simulink model "framework_sim"  (R2019b)
settings: Solver=FixedStepDiscrete  StartTime=T0  StopTime=Tf  FixedStep=Ts  EnableMultiTasking=on
model workspace (MAT data in the model file):
  aKalman : Simulink.Parameter (value not decoded)
  slipEnabler : Simulink.Parameter (value not decoded)
values from neighbouring files (symbols this model uses):
  enable_onlinePlots = 0    [main_framework.m]
  enable_zoom = 0    [main_framework.m]
  HLP_sampleTime = planner.replan_time    [main_framework.m]
  Kb = 10    [main_framework.m]
  Kd_vals = PID_Gain_Scheduling(:,4)    [main_framework.m]
  Ki_vals = PID_Gain_Scheduling(:,3)    [main_framework.m]
  Kp_vals = PID_Gain_Scheduling(:,2)    [main_framework.m]
  latContr_select = 4    [select_lateralController.m]
  mapObjects = scenario.scenario_data.mapObjects    [main_framework.m]
  N_vals = PID_Gain_Scheduling(:,5)    [main_framework.m]
  refRoute_fewPoints = referencePath_fewPoints.refRoute_fewPoints    [main_framework.m]    (also in refPath_poses_fewPoints.mat = [5 34.9682620653 63.3276365473 92.153562059 121.414282249 15; routePlanner.m = [x_cloth_refPath_fewPoints',y_cloth_refPath_fewPoints',theta)
  speed_vals_PID_sched = PID_Gain_Scheduling(:,1)    [main_framework.m]
  tau_D = vehicle_data.steering_system.tau_D    [dataAnalysis.m]    (also in main_framework.m)
  Ts = simulationPars.times.step_size    [main_framework.m]
  vehicle_data = getVehicleDataStruct()    [aeroModel.m]    (also in loadInitialConditions.m; longitSlipModel.m; main_framework.m; perfectAcker.m)
  X0 = loadInitialConditions    [main_framework.m]
undefined symbols (not defined in the file or in its folder): DiscIntNeverNeededParam, loadInitialPose
libraries: simulink_extras x16, drivingvehiclecontroller x2, simulink x1
(part 2 of 3)

== matlab function framework_sim/Vehicle Model ==
  settings: sampleTime=step_size
  data: X input size=24; dX output size=24; extra_params output size=26; torque_req input size=1; delta_req input
function [dX,extra_params] = Vehicle_model(X,torque_req,delta_req)

% ----------------------------------------------------------------
%% 10 DoF Vehicle Model of Formula SAE electric vehicle (Chimera Evoluzione)
%  author: Mattia Piccinini
%  email:  mattia.piccinini@unitn.it
%  date:   18/11/2019
%  The model is partly based on previous work done by Prof. F. Biral and
%  PhD students E. Pagot and L. De Pascali
% ----------------------------------------------------------------


% ----------------------------------------------------------------
%% INPUTS OF THE MODEL
% ----------------------------------------------------------------

% Model inputs are: 
%       - requested actuation torque torque_req in [Nm] (referred to electric 
%           motors if >0 and referred to the braking system if <0)
%       - requested steering angle at the steering wheel delta_req (in [rad])

% Classify the requested actuation torque on the basis of its sign, using 
% regularized positive and negative part functions to distinguish motor
% and braking torques
Tm_req = posPart(torque_req);
Tb_req = -negPart(torque_req);


% ----------------------------------------------------------------
%% OUTPUTS OF THE MODEL
% ----------------------------------------------------------------

% The outputs of the model are the derivatives of all vehicle states,
% collected in the dX vector, as well as some other useful extra parameters 
% to describe vehicle behavior, saved in the extra_params vector

% Empty output vectors are here initialized 
dX = zeros(24,1);  
extra_params = zeros(26,1);  


% ----------------------------------------------------------------
%% STATES OF THE MODEL
% ----------------------------------------------------------------

% The model has 24 states, collected in the X vector

u         = X(1);       % [m/s] vehicle longitudinal speed
v         = X(2);       % [m/s] vehicle lateral speed
z         = X(3);       % [m] vehicle heave (vertical movement of CoM)
Omega     = X(4);       % [rad/s] yaw rate
phi       = X(5);       % [rad] roll angle
mu        = X(6);       % [rad] pitch angle
delta     = X(7);       % [rad] steering angle (at the wheel)
alpha__rr = X(8);       % [rad] side slip angle rear right wheel
alpha__rl = X(9);       % [rad] side slip angle rear left wheel
alpha__fr = X(10);      % [rad] side slip angle front right wheel
alpha__fl = X(11);      % [rad] side slip angle front left wheel
kappa__rr = X(12);      % [-] longitudinal slip rear right wheel
kappa__rl = X(13);      % [-] longitudinal slip rear left wheel
kappa__fr = X(14);      % [-] longitudinal slip front right wheel
kappa__fl = X(15);      % [-] longitudinal slip front left wheel
omega__rr = X(16);      % [rad/s] rotational speed rear right wheel
omega__rl = X(17);      % [rad/s] rotational speed rear left wheel 
omega__fr = X(18);      % [rad/s] rotational speed front right wheel 
omega__fl = X(19);      % [rad/s] rotational speed front left wheel 
z__dot    = X(20);      % [m/s] heave rate of change
phi__dot  = X(21);      % [rad/s] roll angle rate of change
mu__dot   = X(22);      % [rad/s] pitch angle rate of change
Tm        = X(23);      % [Nm] motor torque (same for both rear motors)
Tb        = X(24);      % [Nm] brake torque (same for each wheel)


% ----------------------------------------------------------------
%% VEHICLE DATA AND PARAMETERS
% ----------------------------------------------------------------

% Load a struct containing vehicle parameters. 
% For the meaning of each parameter, refer to the file getVehicleDataStruct
params = getVehicleDataStruct; 

% ----------------------
% SUSPENSION DATA
% ----------------------
% REAR
h__rc_r =  params.rear_suspension.h_rc_r;
% FRONT
h__rc_f =  params.front_suspension.h_rc_f;

% ----------------------                                              
% CHASSIS DATA
% ----------------------
is__xx = params.chassis.is_xx;
is__yy = params.chassis.is_yy;
is__zz = params.chassis.is_zz;
is__xz = params.chassis.is_xz;

% ----------------------
% UNSPRUNG MASS DATA
% ----------------------
% REAR
Rr = params.rear_wheel.Rr;                   
iwa__r = params.rear_wheel.iwa_r;
iwa__f = iwa__r;
% FRONT
Rf = params.front_wheel.Rf;                         

% ----------------------
% OVERALL VEHICLE DATA
% ----------------------
Lf = params.vehicle.Lf;        
Lr = params.vehicle.Lr;             
h__Gs = params.vehicle.hGs;      
Wf = params.vehicle.Wf;    
Wr = params.vehicle.Wr;    
lx = params.vehicle.lx;
ly = params.vehicle.ly;
z__static = h__rc_f + Lf * ((h__rc_r - h__rc_f)/(Lf+Lr));
% Inertia and mass
m = params.vehicle.m;  
ms = params.vehicle.ms;
g = params.vehicle.g;     
i__zz = params.vehicle.i_zz;
i__xz = params.vehicle.i_xz;

% ----------------------
% STEERING SYSTEM DATA        
% ----------------------
tau__D = params.steering_system.tau_D;             
tau__H = params.steering_system.tau_H;   

% ----------------------
% TRANSMISSION DATA
% ----------------------
tau_red = params.transmission.tau_red; 
eff_red = params.transmission.eff_red;

% ----------------------
% MOTOR AND BRAKE ACTUATION DATA
% ----------------------
tau_mot = params.motor.tau_mot;
tau_br  = params.braking.tau_br;


% ----------------------------------------------------------------
%% AUXILIARY MODELS
% ----------------------------------------------------------------

% ----------------------
% MOTOR MODEL
% ----------------------
% Driving torques at the wheels
Tw__rr_traction = MotorModel(Tm,omega__rr,tau_red,eff_red);
Tw__rl_traction = MotorModel(Tm,omega__rl,tau_red,eff_red);
 
% ----------------------
% BRAKE MODEL
% ----------------------
% Rear wheels braking model
[Tw__rr_brake,Tw__rl_brake] = brakeModelRear(Tb,Tb,omega__rr,omega__rl); 
% Front wheels braking model
[Tw__fr_brake,Tw__fl_brake] = brakeModelFront(Tb,Tb,omega__fr,omega__fl);

% ----------------------
% WHEEL TORQUES
% ----------------------
% The total torque for each wheel is the algebraic sum of motor and brake torques
Tw__rr = Tw__rr_traction + Tw__rr_brake;
Tw__rl = Tw__rl_traction + Tw__rl_brake;
Tw__fr = Tw__fr_brake;
Tw__fl = Tw__fl_brake;

% ----------------------
% CAMBER MODEL
% ----------------------
% Static camber + camber gain model, as a function of roll angle phi
[gamma__rr, gamma__rl, gamma__fr, gamma__fl] = camberModel(phi);

% ----------------------
% ACKERMANN STEERING MODEL
% ----------------------
% Compute steering angles for front wheels, with perfect Ackerman steering model
[delta__fr, delta__fl] = perfectAcker(delta);

% ----------------------
% VERTICAL TIRE FORCES MODEL
% ----------------------
% Compute vertical tire loads
VerticalForces = LoadTransferModel(z,phi,mu,z__dot,phi__dot,mu__dot,Omega,u);
Fz__rr = VerticalForces.Fz_rr;
Fz__rl = VerticalForces.Fz_rl;
Fz__fr = VerticalForces.Fz_fr;
Fz__fl = VerticalForces.Fz_fl;

% ----------------------
% LONGITUDINAL SLIPS
% ----------------------
% Longitudinal slip model including a correction for low speed 
[kappa__rr_corr,kappa__rl_corr,kappa__fr_corr,kappa__fl_corr] = longitSlipModel(u,Omega,kappa__rr,kappa__rl,kappa__fr,kappa__fl,omega__rr,omega__rl,omega__fr,omega__fl,delta__fr,delta__fl,Fz__rr,Fz__rl,Fz__fr,Fz__fl,gamma__rr,gamma__rl,gamma__fr,gamma__fl,loadPacejkaParam);

% ----------------------
% AERODYNAMIC MODEL
% ----------------------
% Aero drag, downforce at rear axle, downforce at front axle
[FAxc, FAz__r, FAz__f] = aeroModel(u);
          
% ----------------------
% TIRE PACEJKA MODEL
% ----------------------
% Ensure symmetric behavior of left and right tires by calculating the
% forces and moments for left tires via a previous change of sign of the
% side slip alpha and the camber gamma
[Fx__rr,Fy__rr,AM__rr] = pacejka_model(kappa__rr_corr,Fz__rr,alpha__rr,gamma__rr,loadPacejkaParam);
[Fx__rl,Fy__rl,AM__rl] = pacejka_model(kappa__rl_corr,Fz__rl,-alpha__rl,-gamma__rl,loadPacejkaParam);
[Fx__fr,Fy__fr,AM__fr] = pacejka_model(kappa__fr_corr,Fz__fr,alpha__fr,gamma__fr,loadPacejkaParam);
[Fx__fl,Fy__fl,AM__fl] = pacejka_model(kappa__fl_corr,Fz__fl,-alpha__fl,-gamma__fl,loadPacejkaParam);
% Now perform a second change of sign in order to restore the correct operating conditions
Fy__rl = -Fy__rl; AM__rl = -AM__rl;
Fy__fl = -Fy__fl; AM__fl = -AM__fl;

% ----------------------
% STEADY STATE LONGITUDINAL SLIPS
% ----------------------
[kappa__rr_ss,kappa__rl_ss,kappa__fr_ss,kappa__fl_ss] = steadyStateLongSlips(omega__rr,omega__rl,omega__fr,omega__fl,Omega,u,delta__fr,delta__fl);


% ----------------------------------------------------------------
%% VEHICLE MODEL DIFFERENTIAL EQUATIONS
% ----------------------------------------------------------------

% The following system of ODE is imported from Maple symbolic model

% 3 Newton equations
u_Dot        = ((2 * is__xz * ((is__xx - is__yy - is__zz) * Omega ^ 2 + (h__Gs - z__static) * (-m * g + g * ms - FAz__f - FAz__r + Fz__fl + Fz__fr + Fz__rl + Fz__rr)) * (h__Gs - z__static) * (ms * (h__Gs - z__static) * (ms - m) * z - z__static * (h__Gs - z__static) * ms ^ 2 + m * z__static * (h__Gs - z__static) * ms - m * (is__xx + is__zz)) * ms * mu ^ 2) + ((2 * is__xz * (h__Gs - z__static) ^ 2 * (v * (ms - m) * Omega + delta__fl * Fy__fl + delta__fr * Fy__fr - Fx__fl - Fx__fr - Fx__rl - Fx__rr) * (ms - m) * ms ^ 2 * z ^ 2) + 0.2e1 * (((h__Gs - z__static) * (i__xz * is__xz + i__zz * (is__xx - is__yy - is__zz)) * (ms - m) * ms * Omega ^ 2) - ((ms ^ 2 * is__zz * u * (h__Gs - z__static) ^ 2 * phi) + 0.2e1 * is__xz * (-(ms * iwa__f * omega__fl * (h__Gs - z__static) * delta__fl) / 0.2e1 - (ms * iwa__f * omega__fr * (h__Gs - z__static) * delta__fr) / 0.2e1 + ((z__static * (h__Gs - z__static) * ms ^ 2) - (m * z__static * (h__Gs - z__static) * ms) + (m * (is__xx + is__yy + is__zz)) / 0.2e1) * v + (ms * phi__dot * (is__xx - is__yy - is__zz) * (h__Gs - z__static)) / 0.2e1)) * (ms - m) * Omega + (is__xz * Fy__fl * ((h__Gs - z__static) * (h__Gs - 2 * z__static) * ms ^ 2 + (-h__Gs ^ 2 * m + 3 * h__Gs * m * z__static - 2 * m * z__static ^ 2 + is__yy) * ms - m * (is__xx + is__yy + is__zz)) * delta__fl) + (is__xz * Fy__fr * ((h__Gs - z__static) * (h__Gs - 2 * z__static) * ms ^ 2 + (-h__Gs ^ 2 * m + 3 * h__Gs * m * z__static - 2 * m * z__static ^ 2 + is__yy) * ms - m * (is__xx + is__yy + is__zz)) * delta__fr) - is__xz * (((h__Gs - z__static) * (h__Gs - 2 * z__static - Rf) * ms ^ 2) + (-(2 * m * z__static ^ 2) + 0.3e1 * (h__Gs - Rf / 0.3e1) * m * z__static - (h__Gs * (h__Gs - Rf) * m) + is__yy) * ms - (m * (is__xx + is__yy + is__zz))) * Fx__fl - is__xz * (((h__Gs - z__static) * (h__Gs - 2 * z__static - Rf) * ms ^ 2) + (-(2 * m * z__static ^ 2) + 0.3e1 * (h__Gs - Rf / 0.3e1) * m * z__static - (h__Gs * (h__Gs - Rf) * m) + is__yy) * ms - (m * (is__xx + is__yy + is__zz))) * Fx__fr - is__xz * (((h__Gs - z__static) * (h__Gs - 2 * z__static - Rr) * ms ^ 2) + (-(2 * m * z__static ^ 2) + 0.3e1 * (h__Gs - Rr / 0.3e1) * m * z__static - (h__Gs * (h__Gs - Rr) * m) + is__yy) * ms - (m * (is__xx + is__yy + is__zz))) * Fx__rl - is__xz * (((h__Gs - z__static) * (h__Gs - 2 * z__static - Rr) * ms ^ 2) + (-(2 * m * z__static ^ 2) + 0.3e1 * (h__Gs - Rr / 0.3e1) * m * z__static - (h__Gs * (h__Gs - Rr) * m) + is__yy) * ms - (m * (is__xx + is__yy + is__zz))) * Fx__rr + ((ms - m) * (ms * (h__Gs - z__static) * (-Lf * is__xz + h__Gs * i__zz - i__zz * z__static) * Fz__fl + ms * (h__Gs - z__static) * (-Lf * is__xz + h__Gs * i__zz - i__zz * z__static) * Fz__fr + ms * (h__Gs - z__static) * (Lr * is__xz + h__Gs * i__zz - i__zz * z__static) * Fz__rl + ms * (h__Gs - z__static) * (Lr * is__xz + h__Gs * i__zz - i__zz * z__static) * Fz__rr - ms * (h__Gs - z__static) * (-Lf * is__xz + h__Gs * i__zz - i__zz * z__static) * FAz__f - ms * (h__Gs - z__static) * (Lr * is__xz + h__Gs * i__zz - i__zz * z__static) * FAz__r + ((h__Gs - z__static) ^ 2 * ms + is__yy) * is__xz * FAxc + (-is__xz * Tw__fl - is__xz * Tw__fr - is__xz * Tw__rl - is__xz * Tw__rr + g * i__zz * (h__Gs - z__static) * (ms - m)) * (h__Gs - z__static) * ms))) * (h__Gs - z__static) * ms * z - (2 * (h__Gs - z__static) * ((h__Gs - z__static) * z__static * (i__xz * is__xz + i__zz * (is__xx - is__yy - is__zz)) * ms ^ 2 - (h__Gs - z__static) * z__static * (i__xz * is__xz + i__zz * (is__xx - is__yy - is__zz)) * m * ms + (i__xz * (is__yy + 2 * is__zz) * is__xz + i__zz * is__xx * (is__xx - is__yy - is__zz)) * m) * ms * Omega ^ 2) + ((2 * (h__Gs - z__static) ^ 2 * is__zz * u * (z__static * (h__Gs - z__static) * ms ^ 2 - m * z__static * (h__Gs - z__static) * ms + is__xx * m) * ms ^ 2 * phi + 2 * is__xz * (-ms * iwa__f * omega__fl * (h__Gs - z__static) * delta__fl - ms * iwa__f * omega__fr * (h__Gs - z__static) * delta__fr + (z__static * (h__Gs - z__static) * ms ^ 2 - m * z__static * (h__Gs - z__static) * ms + is__yy * m) * v + ms * phi__dot * (is__xx - is__yy - is__zz) * (h__Gs - z__static)) * (z__static * (h__Gs - z__static) * ms ^ 2 - m * z__static * (h__Gs - z__static) * ms + m * (is__xx + is__zz))) * Omega) - (2 * ((h__Gs - z__static) ^ 2 * ms + is__yy) * is__xz * Fy__fl * (z__static * (h__Gs - z__static) * ms ^ 2 - m * z__static * (h__Gs - z__static) * ms + m * (is__xx + is__zz)) * delta__fl) - (2 * ((h__Gs - z__static) ^ 2 * ms + is__yy) * is__xz * Fy__fr * (z__static * (h__Gs - z__static) * ms ^ 2 - m * z__static * (h__Gs - z__static) * ms + m * (is__xx + is__zz)) * delta__fr) + (2 * ((h__Gs - z__static) * (h__Gs - z__static - Rf) * ms + is__yy) * is__xz * (z__static * (h__Gs - z__static) * ms ^ 2 - m * z__static * (h__Gs - z__static) * ms + m * (is__xx + is__zz)) * Fx__fl) + (2 * ((h__Gs - z__static) * (h__Gs - z__static - Rf) * ms + is__yy) * is__xz * (z__static * (h__Gs - z__static) * ms ^ 2 - m * z__static * (h__Gs - z__static) * ms + m * (is__xx + is__zz)) * Fx__fr) + (2 * is__xz * ((h__Gs - z__static) * (h__Gs - z__static - Rr) * ms + is__yy) * (z__static * (h__Gs - z__static) * ms ^ 2 - m * z__static * (h__Gs - z__static) * ms + m * (is__xx + is__zz)) * Fx__rl) + (2 * is__xz * ((h__Gs - z__static) * (h__Gs - z__static - Rr) * ms + is__yy) * (z__static * (h__Gs - z__static) * ms ^ 2 - m * z__static * (h__Gs - z__static) * ms + m * (is__xx + is__zz)) * Fx__rr) - (2 * (h__Gs - z__static) * (z__static * (h__Gs - z__static) * (-Lf * is__xz + h__Gs * i__zz - i__zz * z__static) * ms ^ 2 - m * z__static * (h__Gs - z__static) * (-Lf * is__xz + h__Gs * i__zz - i__zz * z__static) * ms - m * ((-i__xz * is__xz + i__zz * is__xx) * z__static + (i__xz * is__xz - i__zz * is__xx) * h__Gs + is__xz * Lf * (is__xx + is__zz))) * ms * Fz__fl) - (2 * (h__Gs - z__static) * (z__static * (h__Gs - z__static) * (-Lf * is__xz + h__Gs * i__zz - i__zz * z__static) * ms ^ 2 - m * z__static * (h__Gs - z__static) * (-Lf * is__xz + h__Gs * i__zz - i__zz * z__static) * ms - m * ((-i__xz * is__xz + i__zz * is__xx) * z__static + (i__xz * is__xz - i__zz * is__xx) * h__Gs + is__xz * Lf * (is__xx + is__zz))) * ms * Fz__fr) - (2 * (z__static * (h__Gs - z__static) * (Lr * is__xz + h__Gs * i__zz - i__zz * z__static) * ms ^ 2 - m * z__static * (h__Gs - z__static) * (Lr * is__xz + h__Gs * i__zz - i__zz * z__static) * ms - ((-i__xz * is__xz + i__zz * is__xx) * z__static + (i__xz * is__xz - i__zz * is__xx) * h__Gs - is__xz * Lr * (is__xx + is__zz)) * m) * (h__Gs - z__static) * ms * Fz__rl) - (2 * (z__static * (h__Gs - z__static) * (Lr * is__xz + h__Gs * i__zz - i__zz * z__static) * ms ^ 2 - m * z__static * (h__Gs - z__static) * (Lr * is__xz + h__Gs * i__zz - i__zz * z__static) * ms - ((-i__xz * is__xz + i__zz * is__xx) * z__static + (i__xz * is__xz - i__zz * is__xx) * h__Gs - is__xz * Lr * (is__xx + is__zz)) * m) * (h__Gs - z__static) * ms * Fz__rr) + (2 * (h__Gs - z__static) * (z__static * (h__Gs - z__static) * (-Lf * is__xz + h__Gs * i__zz - i__zz * z__static) * ms ^ 2 - m * z__static * (h__Gs - z__static) * (-Lf * is__xz + h__Gs * i__zz - i__zz * z__static) * ms - m * ((-i__xz * is__xz + i__zz * is__xx) * z__static + (i__xz * is__xz - i__zz * is__xx) * h__Gs + is__xz * Lf * (is__xx + is__zz))) * ms * FAz__f) + (2 * (z__static * (h__Gs - z__static) * (Lr * is__xz + h__Gs * i__zz - i__zz * z__static) * ms ^ 2 - m * z__static * (h__Gs - z__static) * (Lr * is__xz + h__Gs * i__zz - i__zz * z__static) * ms - ((-i__xz * is__xz + i__zz * is__xx) * z__static + (i__xz * is__xz - i__zz * is__xx) * h__Gs - is__xz * Lr * (is__xx + is__zz)) * m) * (h__Gs - z__static) * ms * FAz__r) - (2 * ((h__Gs - z__static) ^ 2 * ms + is__yy) * is__xz * (z__static * (h__Gs - z__static) * ms ^ 2 - m * z__static * (h__Gs - z__static) * ms + m * (is__xx + is__zz)) * FAxc) - (2 * (-is__xz * (z__static * (h__Gs - z__static) * ms ^ 2 - m * z__static * (h__Gs - z__static) * ms + m * (is__xx + is__zz)) * Tw__fl - is__xz * (z__static * (h__Gs - z__static) * ms ^ 2 - m * z__static * (h__Gs - z__static) * ms + m * (is__xx + is__zz)) * Tw__fr - is__xz * (z__static * (h__Gs - z__static) * ms ^ 2 - m * z__static * (h__Gs - z__static) * ms + m * (is__xx + is__zz)) * Tw__rl - is__xz * (z__static * (h__Gs - z__static) * ms ^ 2 - m * z__static * (h__Gs - z__static) * ms + m * (is__xx + is__zz)) * Tw__rr + (h__Gs - z__static) * (ms - m) * g * (i__zz * z__static * (h__Gs - z__static) * ms ^ 2 - i__zz * m * z__static * (h__Gs - z__static) * ms - m * (i__xz * is__xz - i__zz * is__xx))) * (h__Gs - z__static) * ms)) * mu + (2 * (h__Gs - z__static) ^ 2 * (v * (ms - m) * Omega + delta__fl * Fy__fl + delta__fr * Fy__fr - Fx__fl - Fx__fr - Fx__rl - Fx__rr) * (ms - m) * i__zz * ms ^ 2 * z ^ 2) - 0.4e1 * (h__Gs - z__static) * (-(ms * (is__xz * is__zz * phi ^ 2 + i__xz * i__zz) * (h__Gs - z__static) * (ms - m) * Omega ^ 2) / 0.2e1 + (-(ms * i__zz * iwa__f * omega__fl * (h__Gs - z__static) * delta__fl) / 0.2e1 - (ms * i__zz * iwa__f * omega__fr * (h__Gs - z__static) * delta__fr) / 0.2e1 + ((i__zz * z__static * (h__Gs - z__static) * ms ^ 2) - (i__zz * m * z__static * (h__Gs - z__static) * ms) - ((i__xz * is__xz - i__zz * (is__xx + is__yy)) * m) / 0.2e1) * v + (ms * i__zz * phi__dot * (is__xx - is__yy - is__zz) * (h__Gs - z__static)) / 0.2e1) * (ms - m) * Omega - ((((Lf * (h__Gs - z__static) * ms - h__Gs * m * Lf + m * z__static * Lf - is__xz) * Fx__fl) + (Fy__fl * Wf * (h__Gs - z__static) * (ms - m)) / 0.2e1) * delta__fl + (((Lf * (h__Gs - z__static) * ms - h__Gs * m * Lf + m * z__static * Lf - is__xz) * Fx__fr) - (Fy__fr * Wf * (h__Gs - z__static) * (ms - m)) / 0.2e1) * delta__fr - (Wf * (h__Gs - z__static) * (ms - m) * Fx__fl) / 0.2e1 + (Wf * (h__Gs - z__static) * (ms - m) * Fx__fr) / 0.2e1 - (Wr * (h__Gs - z__static) * (ms - m) * Fx__rl) / 0.2e1 + (Wr * (h__Gs - z__static) * (ms - m) * Fx__rr) / 0.2e1 + ((Lf * (h__Gs - z__static) * ms - h__Gs * m * Lf + m * z__static * Lf - is__xz) * Fy__fl) + ((Lf * (h__Gs - z__static) * ms - h__Gs * m * Lf + m * z__static * Lf - is__xz) * Fy__fr) + ((-Lr * (h__Gs - z__static) * ms + h__Gs * m * Lr - m * z__static * Lr - is__xz) * Fy__rl) + ((-Lr * (h__Gs - z__static) * ms + h__Gs * m * Lr - m * z__static * Lr - is__xz) * Fy__rr) + ((AM__fl + AM__fr + AM__rl + AM__rr) * (h__Gs - z__static) * (ms - m))) * is__zz * ms * phi / 0.2e1 - (Fy__fl * (i__zz * (h__Gs - z__static) * (h__Gs - 2 * z__static) * ms ^ 2 - i__zz * (h__Gs ^ 2 * m - 3 * h__Gs * m * z__static + 2 * m * z__static ^ 2 - is__yy) * ms + (i__xz * is__xz - i__zz * (is__xx + is__yy)) * m) * delta__fl) / 0.2e1 - (Fy__fr * (i__zz * (h__Gs - z__static) * (h__Gs - 2 * z__static) * ms ^ 2 - i__zz * (h__Gs ^ 2 * m - 3 * h__Gs * m * z__static + 2 * m * z__static ^ 2 - is__yy) * ms + (i__xz * is__xz - i__zz * (is__xx + is__yy)) * m) * delta__fr) / 0.2e1 + ((i__zz * (h__Gs - z__static) * (h__Gs - 2 * z__static - Rf) * ms ^ 2) / 0.2e1 - ((2 * m * z__static ^ 2) - 0.3e1 * (h__Gs - Rf / 0.3e1) * m * z__static + (h__Gs * (h__Gs - Rf) * m) - is__yy) * i__zz * ms / 0.2e1 + ((i__xz * is__xz - i__zz * (is__xx + is__yy)) * m) / 0.2e1) * Fx__fl + ((i__zz * (h__Gs - z__static) * (h__Gs - 2 * z__static - Rf) * ms ^ 2) / 0.2e1 - ((2 * m * z__static ^ 2) - 0.3e1 * (h__Gs - Rf / 0.3e1) * m * z__static + (h__Gs * (h__Gs - Rf) * m) - is__yy) * i__zz * ms / 0.2e1 + ((i__xz * is__xz - i__zz * (is__xx + is__yy)) * m) / 0.2e1) * Fx__fr + ((i__zz * (h__Gs - z__static) * (h__Gs - 2 * z__static - Rr) * ms ^ 2) / 0.2e1 - ((2 * m * z__static ^ 2) - 0.3e1 * (h__Gs - Rr / 0.3e1) * m * z__static + (h__Gs * (h__Gs - Rr) * m) - is__yy) * i__zz * ms / 0.2e1 + ((i__xz * is__xz - i__zz * (is__xx + is__yy)) * m) / 0.2e1) * Fx__rl + ((i__zz * (h__Gs - z__static) * (h__Gs - 2 * z__static - Rr) * ms ^ 2) / 0.2e1 - ((2 * m * z__static ^ 2) - 0.3e1 * (h__Gs - Rr / 0.3e1) * m * z__static + (h__Gs * (h__Gs - Rr) * m) - is__yy) * i__zz * ms / 0.2e1 + ((i__xz * is__xz - i__zz * (is__xx + is__yy)) * m) / 0.2e1) * Fx__rr - ((ms - m) * i__zz * (-Lf * (h__Gs - z__static) * ms * Fz__fl - Lf * (h__Gs - z__static) * ms * Fz__fr + Lr * (h__Gs - z__static) * ms * Fz__rl + Lr * (h__Gs - z__static) * ms * Fz__rr + Lf * (h__Gs - z__static) * ms * FAz__f - Lr * (h__Gs - z__static) * ms * FAz__r + ((h__Gs - z__static) ^ 2 * ms + is__yy) * FAxc - ms * (Tw__fl + Tw__fr + Tw__rl + Tw__rr) * (h__Gs - z__static))) / 0.2e1) * ms * z - (2 * (h__Gs - z__static) * ((z__static * (h__Gs - z__static) * ms ^ 2 - m * z__static * (h__Gs - z__static) * ms + m * (is__yy - is__zz)) * is__xz * is__zz * phi ^ 2 + i__xz * (i__zz * z__static * (h__Gs - z__static) * ms ^ 2 - i__zz * m * z__static * (h__Gs - z__static) * ms - m * (i__xz * is__xz - i__zz * is__xx))) * ms * Omega ^ 2) + ((2 * is__xz * (h__Gs - z__static) * (-iwa__f * omega__fl - iwa__f * omega__fr + (is__xx - is__yy + is__zz) * mu__dot - iwa__r * (omega__rl + omega__rr)) * is__zz * m * ms * phi + 2 * (-ms * iwa__f * omega__fl * (h__Gs - z__static) * delta__fl - ms * iwa__f * omega__fr * (h__Gs - z__static) * delta__fr + (z__static * (h__Gs - z__static) * ms ^ 2 - m * z__static * (h__Gs - z__static) * ms + is__yy * m) * v + ms * phi__dot * (is__xx - is__yy - is__zz) * (h__Gs - z__static)) * (i__zz * z__static * (h__Gs - z__static) * ms ^ 2 - i__zz * m * z__static * (h__Gs - z__static) * ms - m * (i__xz * is__xz - i__zz * is__xx))) * Omega) - (2 * ms * is__xz * is__zz * m * (h__Gs - z__static) ^ 2 * (-m * g + g * ms - FAz__f - FAz__r + Fz__fl + Fz__fr + Fz__rl + Fz__rr) * phi ^ 2) - 0.2e1 * (h__Gs - z__static) * ((((z__static * Lf * (h__Gs - z__static) * ms ^ 2 - z__static * (h__Gs * m * Lf - m * z__static * Lf + is__xz) * ms + m * (is__xx * Lf - is__xz * Rf + h__Gs * is__xz)) * Fx__fl) + (Wf * (z__static * (h__Gs - z__static) * ms ^ 2 - m * z__static * (h__Gs - z__static) * ms + is__xx * m) * Fy__fl) / 0.2e1 + (is__xz * m * Tw__fl)) * delta__fl + (((z__static * Lf * (h__Gs - z__static) * ms ^ 2 - z__static * (h__Gs * m * Lf - m * z__static * Lf + is__xz) * ms + m * (is__xx * Lf - is__xz * Rf + h__Gs * is__xz)) * Fx__fr) - (Wf * (z__static * (h__Gs - z__static) * ms ^ 2 - m * z__static * (h__Gs - z__static) * ms + is__xx * m) * Fy__fr) / 0.2e1 + (is__xz * m * Tw__fr)) * delta__fr - (Wf * (z__static * (h__Gs - z__static) * ms ^ 2 - m * z__static * (h__Gs - z__static) * ms + is__xx * m) * Fx__fl) / 0.2e1 + (Wf * (z__static * (h__Gs - z__static) * ms ^ 2 - m * z__static * (h__Gs - z__static) * ms + is__xx * m) * Fx__fr) / 0.2e1 - (Wr * (z__static * (h__Gs - z__static) * ms ^ 2 - m * z__static * (h__Gs - z__static) * ms + is__xx * m) * Fx__rl) / 0.2e1 + (Wr * (z__static * (h__Gs - z__static) * ms ^ 2 - m * z__static * (h__Gs - z__static) * ms + is__xx * m) * Fx__rr) / 0.2e1 + ((z__static * Lf * (h__Gs - z__static) * ms ^ 2 - z__static * (h__Gs * m * Lf - m * z__static * Lf + is__xz) * ms + m * (is__xx * Lf + h__Gs * is__xz)) * Fy__fl) + ((z__static * Lf * (h__Gs - z__static) * ms ^ 2 - z__static * (h__Gs * m * Lf - m * z__static * Lf + is__xz) * ms + m * (is__xx * Lf + h__Gs * is__xz)) * Fy__fr) + (is__xz * m * Fz__fl * Wf) / 0.2e1 - (is__xz * m * Fz__fr * Wf) / 0.2e1 + (is__xz * m * Fz__rl * Wr) / 0.2e1 - (is__xz * m * Fz__rr * Wr) / 0.2e1 + ((-Lr * z__static * (h__Gs - z__static) * ms ^ 2 + z__static * (h__Gs * m * Lr - m * z__static * Lr - is__xz) * ms + m * (-Lr * is__xx + h__Gs * is__xz)) * Fy__rl) + ((-Lr * z__static * (h__Gs - z__static) * ms ^ 2 + z__static * (h__Gs * m * Lr - m * z__static * Lr - is__xz) * ms + m * (-Lr * is__xx + h__Gs * is__xz)) * Fy__rr) + ((AM__fl + AM__fr + AM__rl + AM__rr) * (z__static * (h__Gs - z__static) * ms ^ 2 - m * z__static * (h__Gs - z__static) * ms + is__xx * m))) * is__zz * ms * phi - (2 * (((h__Gs - z__static) ^ 2 * ms + is__yy) * Fy__fl * delta__fl + ((h__Gs - z__static) ^ 2 * ms + is__yy) * Fy__fr * delta__fr + (-(h__Gs - z__static) * (h__Gs - z__static - Rf) * ms - is__yy) * Fx__fl + (-(h__Gs - z__static) * (h__Gs - z__static - Rf) * ms - is__yy) * Fx__fr + (-(h__Gs - z__static) * (h__Gs - z__static - Rr) * ms - is__yy) * Fx__rl + (-(h__Gs - z__static) * (h__Gs - z__static - Rr) * ms - is__yy) * Fx__rr - Lf * (h__Gs - z__static) * ms * Fz__fl - Lf * (h__Gs - z__static) * ms * Fz__fr + Lr * (h__Gs - z__static) * ms * Fz__rl + Lr * (h__Gs - z__static) * ms * Fz__rr + Lf * (h__Gs - z__static) * ms * FAz__f - Lr * (h__Gs - z__static) * ms * FAz__r + ((h__Gs - z__static) ^ 2 * ms + is__yy) * FAxc - ms * (Tw__fl + Tw__fr + Tw__rl + Tw__rr) * (h__Gs - z__static)) * (i__zz * z__static * (h__Gs - z__static) * ms ^ 2 - i__zz * m * z__static * (h__Gs - z__static) * ms - m * (i__xz * is__xz - i__zz * is__xx)))) / (2 * (ms * (h__Gs - z__static) * (ms - m) * z - z__static * (h__Gs - z__static) * ms ^ 2 + m * z__static * (h__Gs - z__static) * ms - is__yy * m) * is__xz * (ms * (h__Gs - z__static) * (ms - m) * z - z__static * (h__Gs - z__static) * ms ^ 2 + m * z__static * (h__Gs - z__static) * ms - m * (is__xx + is__zz)) * mu + 2 * ms ^ 2 * i__zz * (h__Gs - z__static) ^ 2 * (ms - m) ^ 2 * z ^ 2 + 2 * (h__Gs - z__static) * (ms - m) * (ms ^ 2 * is__zz * (h__Gs - z__static) ^ 2 * phi ^ 2 - 2 * i__zz * z__static * (h__Gs - z__static) * ms ^ 2 + 2 * i__zz * m * z__static * (h__Gs - z__static) * ms + (i__xz * is__xz - i__zz * (is__xx + is__yy)) * m) * ms * z - 2 * (h__Gs - z__static) ^ 2 * is__zz * (z__static * (h__Gs - z__static) * ms ^ 2 - m * z__static * (h__Gs - z__static) * ms + is__xx * m) * ms ^ 2 * phi ^ 2 + 2 * (z__static * (h__Gs - z__static) * ms ^ 2 - m * z__static * (h__Gs - z__static) * ms + is__yy * m) * (i__zz * z__static * (h__Gs - z__static) * ms ^ 2 - i__zz * m * z__static * (h__Gs - z__static) * ms - m * (i__xz * is__xz - i__zz * is__xx)));
v_Dot        = (-(2 * (h__Gs - z__static) ^ 2 * is__zz * ms ^ 2 * (((is__xx - is__yy - is__zz) * Omega ^ 2 + (h__Gs - z__static) * (-m * g + g * ms - FAz__f - FAz__r + Fz__fl + Fz__fr + Fz__rl + Fz__rr)) * (h__Gs - z__static) * ms * phi + (ms * (h__Gs - z__static) * (ms - m) * z - z__static * (h__Gs - z__static) * ms ^ 2 + m * z__static * (h__Gs - z__static) * ms - is__yy * m) * u * Omega) * mu ^ 2) + ((2 * (h__Gs - z__static) * (-(-is__xz * (is__xx - is__yy + 2 * is__zz) * (ms - m) * Omega ^ 2 + ms * is__zz * v * (h__Gs - z__static) * (ms - m) * Omega + (h__Gs - z__static) * (ms * is__zz * Fy__fl * delta__fl + ms * is__zz * Fy__fr * delta__fr - ms * is__zz * Fx__fl - ms * is__zz * Fx__fr + is__xz * (ms - m) * Fz__fl + is__xz * (ms - m) * Fz__fr + is__xz * (ms - m) * Fz__rl + is__xz * (ms - m) * Fz__rr - is__xz * (ms - m) * FAz__f - is__xz * (ms - m) * FAz__r - ms * is__zz * Fx__rl - ms * is__zz * Fx__rr + g * is__xz * (ms - m) ^ 2)) * (h__Gs - z__static) * ms * z + ((h__Gs - z__static) * (((-is__xx + is__yy - 2 * is__zz) * is__xz - i__xz * (is__xx - is__yy - 2 * is__zz)) * z__static + h__Gs * i__xz * (is__xx - is__yy - 2 * is__zz)) * ms ^ 2 + is__xz * m * z__static * (is__xx - is__yy + 2 * is__zz) * (h__Gs - z__static) * ms - is__xz * is__yy * m * (is__xx - is__yy + 2 * is__zz)) * Omega ^ 2 + (h__Gs - z__static) * (-ms * iwa__f * omega__fl * (h__Gs - z__static) * delta__fl - ms * iwa__f * omega__fr * (h__Gs - z__static) * delta__fr + (z__static * (h__Gs - z__static) * ms ^ 2 - m * z__static * (h__Gs - z__static) * ms + is__yy * m) * v + ms * phi__dot * (is__xx - is__yy - is__zz) * (h__Gs - z__static)) * is__zz * ms * Omega + (h__Gs - z__static) * (-((h__Gs - z__static) ^ 2 * ms + is__yy) * Fy__fl * is__zz * ms * delta__fl - ((h__Gs - z__static) ^ 2 * ms + is__yy) * Fy__fr * is__zz * ms * delta__fr + ((h__Gs - z__static) * (h__Gs - z__static - Rf) * ms + is__yy) * is__zz * ms * Fx__fl + ((h__Gs - z__static) * (h__Gs - z__static - Rf) * ms + is__yy) * is__zz * ms * Fx__fr + ((h__Gs - z__static) * ((-i__xz + is__xz) * z__static + h__Gs * i__xz + is__zz * Lf) * ms ^ 2 - is__xz * m * z__static * (h__Gs - z__static) * ms + is__xz * is__yy * m) * Fz__fl + ((h__Gs - z__static) * ((-i__xz + is__xz) * z__static + h__Gs * i__xz + is__zz * Lf) * ms ^ 2 - is__xz * m * z__static * (h__Gs - z__static) * ms + is__xz * is__yy * m) * Fz__fr + ((h__Gs - z__static) * ((-i__xz + is__xz) * z__static + h__Gs * i__xz - is__zz * Lr) * ms ^ 2 - is__xz * m * z__static * (h__Gs - z__static) * ms + is__xz * is__yy * m) * Fz__rl + ((h__Gs - z__static) * ((-i__xz + is__xz) * z__static + h__Gs * i__xz - is__zz * Lr) * ms ^ 2 - is__xz * m * z__static * (h__Gs - z__static) * ms + is__xz * is__yy * m) * Fz__rr + (-(h__Gs - z__static) * ((-i__xz + is__xz) * z__static + h__Gs * i__xz + is__zz * Lf) * ms ^ 2 + is__xz * m * z__static * (h__Gs - z__static) * ms - is__xz * is__yy * m) * FAz__f + (-(h__Gs - z__static) * ((-i__xz + is__xz) * z__static + h__Gs * i__xz - is__zz * Lr) * ms ^ 2 + is__xz * m * z__static * (h__Gs - z__static) * ms - is__xz * is__yy * m) * FAz__r + ((h__Gs - z__static) * (h__Gs - z__static - Rr) * ms + is__yy) * is__zz * ms * Fx__rl + ((h__Gs - z__static) * (h__Gs - z__static - Rr) * ms + is__yy) * is__zz * ms * Fx__rr + ms ^ 2 * is__zz * (h__Gs - z__static) * Tw__fl + ms ^ 2 * is__zz * (h__Gs - z__static) * Tw__fr - ((h__Gs - z__static) ^ 2 * ms + is__yy) * is__zz * ms * FAxc + ms ^ 2 * is__zz * (h__Gs - z__static) * Tw__rl + ms ^ 2 * is__zz * (h__Gs - z__static) * Tw__rr + (ms - m) * ((h__Gs - z__static) * ((-i__xz + is__xz) * z__static + h__Gs * i__xz) * ms ^ 2 - is__xz * m * z__static * (h__Gs - z__static) * ms + is__xz * is__yy * m) * g)) * ms * phi) + 0.2e1 * (ms * (h__Gs - z__static) * (ms - m) * z - z__static * (h__Gs - z__static) * ms ^ 2 + m * z__static * (h__Gs - z__static) * ms - is__yy * m) * (-(is__xz * (h__Gs - z__static) * (u * (ms - m) * Omega + Fx__fl * delta__fl + Fx__fr * delta__fr + Fy__fl + Fy__fr + Fy__rl + Fy__rr) * ms * z) + ((((h__Gs - z__static) * ((-i__xz + is__xz) * z__static + h__Gs * i__xz) * ms ^ 2 - is__xz * m * z__static * (h__Gs - z__static) * ms + is__xz * m * (is__xx + is__zz)) * u + is__xz * (h__Gs - z__static) * (-iwa__f * omega__fl - iwa__f * omega__fr + (is__xx - is__yy + is__zz) * mu__dot - iwa__r * (omega__rl + omega__rr)) * ms) * Omega) + (((-(h__Gs - z__static) * (-is__zz * Lf - is__xz * Rf + h__Gs * is__xz - is__xz * z__static) * ms - is__xz * (is__xx + is__zz)) * Fx__fl) - (h__Gs - z__static) * (-(is__zz * Fy__fl * Wf) / 0.2e1 + (is__xz * Tw__fl)) * ms) * delta__fl + (((-(h__Gs - z__static) * (-is__zz * Lf - is__xz * Rf + h__Gs * is__xz - is__xz * z__static) * ms - is__xz * (is__xx + is__zz)) * Fx__fr) - (h__Gs - z__static) * ((is__zz * Fy__fr * Wf) / 0.2e1 + (is__xz * Tw__fr)) * ms) * delta__fr - (ms * is__zz * Wf * (h__Gs - z__static) * Fx__fl) / 0.2e1 + (ms * is__zz * Wf * (h__Gs - z__static) * Fx__fr) / 0.2e1 + ((-(h__Gs - z__static) * (-is__zz * Lf + h__Gs * is__xz - is__xz * z__static) * ms - is__xz * (is__xx + is__zz)) * Fy__fl) + ((-(h__Gs - z__static) * (-is__zz * Lf + h__Gs * is__xz - is__xz * z__static) * ms - is__xz * (is__xx + is__zz)) * Fy__fr) + ((-(h__Gs - z__static) * (is__zz * Lr + h__Gs * is__xz - is__xz * z__static) * ms - is__xz * (is__xx + is__zz)) * Fy__rl) + ((-(h__Gs - z__static) * (is__zz * Lr + h__Gs * is__xz - is__xz * z__static) * ms - is__xz * (is__xx + is__zz)) * Fy__rr) - (h__Gs - z__static) * ((is__xz * Wf * Fz__fl) - (is__xz * Wf * Fz__fr) + (is__xz * Wr * Fz__rl) - (is__xz * Wr * Fz__rr) - 0.2e1 * (-(Wr * Fx__rl) / 0.2e1 + (Wr * Fx__rr) / 0.2e1 + AM__fl + AM__fr + AM__rl + AM__rr) * is__zz) * ms / 0.2e1)) * mu - (2 * (h__Gs - z__static) ^ 3 * ((-is__xx + is__yy - is__zz) * Omega ^ 2 + (h__Gs - z__static) * (-m * g + g * ms - FAz__f - FAz__r + Fz__fl + Fz__fr + Fz__rl + Fz__rr)) * is__zz * ms ^ 3 * phi ^ 3) - 0.2e1 * ((h__Gs - z__static) ^ 2) * is__zz * (((h__Gs - z__static) * (u * (ms - m) * Omega + Fx__fl * delta__fl + Fx__fr * delta__fr + Fy__fl + Fy__fr + Fy__rl + Fy__rr) * ms * z) + (((-z__static * (h__Gs - z__static) * ms ^ 2 + m * z__static * (h__Gs - z__static) * ms - is__xx * m) * u - (h__Gs - z__static) * (-iwa__f * omega__fl - iwa__f * omega__fr + (is__xx - is__yy + is__zz) * mu__dot - iwa__r * (omega__rl + omega__rr)) * ms) * Omega) + ((((h__Gs - z__static) * (h__Gs - z__static - Rf) * ms + is__xx) * Fx__fl + ms * Tw__fl * (h__Gs - z__static)) * delta__fl) + ((((h__Gs - z__static) * (h__Gs - z__static - Rf) * ms + is__xx) * Fx__fr + ms * Tw__fr * (h__Gs - z__static)) * delta__fr) + (((h__Gs - z__static) ^ 2 * ms + is__xx) * Fy__fl) + (((h__Gs - z__static) ^ 2 * ms + is__xx) * Fy__fr) + (((h__Gs - z__static) ^ 2 * ms + is__xx) * Fy__rl) + (((h__Gs - z__static) ^ 2 * ms + is__xx) * Fy__rr) + ((h__Gs - z__static) * (Wf * Fz__fl - Wf * Fz__fr + Wr * (Fz__rl - Fz__rr)) * ms) / 0.2e1) * (ms ^ 2) * (phi ^ 2) - (2 * (h__Gs - z__static) * ((h__Gs - z__static) * ((ms - m) * (i__xz * is__xz - i__zz * (is__xx - is__yy + is__zz)) * Omega ^ 2 - ms * i__xz * v * (h__Gs - z__static) * (ms - m) * Omega + (h__Gs - z__static) * (-ms * i__xz * Fy__fl * delta__fl - ms * i__xz * Fy__fr * delta__fr + ms * i__xz * Fx__fl + ms * i__xz * Fx__fr + i__zz * (ms - m) * Fz__fl + i__zz * (ms - m) * Fz__fr + i__zz * (ms - m) * Fz__rl + i__zz * (ms - m) * Fz__rr - i__zz * (ms - m) * FAz__f - i__zz * (ms - m) * FAz__r + ms * i__xz * Fx__rl + ms * i__xz * Fx__rr + g * i__zz * (ms - m) ^ 2)) * ms * z + (-(h__Gs - z__static) * ((i__xz * is__xz - i__zz * is__zz + (-is__xx + is__yy) * i__zz - i__xz ^ 2) * z__static + i__xz ^ 2 * h__Gs) * ms ^ 2 + (h__Gs - z__static) * z__static * m * (i__xz * is__xz - i__zz * (is__xx - is__yy + is__zz)) * ms - is__yy * m * (i__xz * is__xz - i__zz * (is__xx - is__yy + is__zz))) * Omega ^ 2 + i__xz * (h__Gs - z__static) * (-ms * iwa__f * omega__fl * (h__Gs - z__static) * delta__fl - ms * iwa__f * omega__fr * (h__Gs - z__static) * delta__fr + (z__static * (h__Gs - z__static) * ms ^ 2 - m * z__static * (h__Gs - z__static) * ms + is__yy * m) * v + ms * phi__dot * (is__xx - is__yy - is__zz) * (h__Gs - z__static)) * ms * Omega - (h__Gs - z__static) * (((h__Gs - z__static) ^ 2 * ms + is__yy) * i__xz * Fy__fl * ms * delta__fl + ((h__Gs - z__static) ^ 2 * ms + is__yy) * i__xz * Fy__fr * ms * delta__fr - ((h__Gs - z__static) * (h__Gs - z__static - Rf) * ms + is__yy) * i__xz * ms * Fx__fl - ((h__Gs - z__static) * (h__Gs - z__static - Rf) * ms + is__yy) * i__xz * ms * Fx__fr + (-(Lf * i__xz - i__zz * z__static) * (h__Gs - z__static) * ms ^ 2 - i__zz * m * z__static * (h__Gs - z__static) * ms + i__zz * is__yy * m) * Fz__fl + (-(Lf * i__xz - i__zz * z__static) * (h__Gs - z__static) * ms ^ 2 - i__zz * m * z__static * (h__Gs - z__static) * ms + i__zz * is__yy * m) * Fz__fr + ((Lr * i__xz + i__zz * z__static) * (h__Gs - z__static) * ms ^ 2 - i__zz * m * z__static * (h__Gs - z__static) * ms + i__zz * is__yy * m) * Fz__rl + ((Lr * i__xz + i__zz * z__static) * (h__Gs - z__static) * ms ^ 2 - i__zz * m * z__static * (h__Gs - z__static) * ms + i__zz * is__yy * m) * Fz__rr + ((Lf * i__xz - i__zz * z__static) * (h__Gs - z__static) * ms ^ 2 + i__zz * m * z__static * (h__Gs - z__static) * ms - i__zz * is__yy * m) * FAz__f + (-(Lr * i__xz + i__zz * z__static) * (h__Gs - z__static) * ms ^ 2 + i__zz * m * z__static * (h__Gs - z__static) * ms - i__zz * is__yy * m) * FAz__r - i__xz * ((h__Gs - z__static) * (h__Gs - z__static - Rr) * ms + is__yy) * ms * Fx__rl - i__xz * ((h__Gs - z__static) * (h__Gs - z__static - Rr) * ms + is__yy) * ms * Fx__rr - ms ^ 2 * i__xz * (h__Gs - z__static) * Tw__fl - ms ^ 2 * i__xz * (h__Gs - z__static) * Tw__fr + ((h__Gs - z__static) ^ 2 * ms + is__yy) * i__xz * ms * FAxc - ms ^ 2 * i__xz * (h__Gs - z__static) * Tw__rl - ms ^ 2 * i__xz * (h__Gs - z__static) * Tw__rr + (ms - m) * i__zz * (z__static * (h__Gs - z__static) * ms ^ 2 - m * z__static * (h__Gs - z__static) * ms + is__yy * m) * g)) * ms * phi) - 0.2e1 * (ms * (h__Gs - z__static) * (ms - m) * z - z__static * (h__Gs - z__static) * ms ^ 2 + m * z__static * (h__Gs - z__static) * ms - is__yy * m) * (((h__Gs - z__static) * (u * (ms - m) * Omega + Fx__fl * delta__fl + Fx__fr * delta__fr + Fy__fl + Fy__fr + Fy__rl + Fy__rr) * i__zz * ms * z) + (((-i__zz * z__static * (h__Gs - z__static) * ms ^ 2 + i__zz * m * z__static * (h__Gs - z__static) * ms + m * (i__xz * is__xz - i__zz * is__xx)) * u - (h__Gs - z__static) * (-iwa__f * omega__fl - iwa__f * omega__fr + (is__xx - is__yy + is__zz) * mu__dot - iwa__r * (omega__rl + omega__rr)) * i__zz * ms) * Omega) + ((((h__Gs - z__static) * (Lf * i__xz - Rf * i__zz + h__Gs * i__zz - i__zz * z__static) * ms - i__xz * is__xz + i__zz * is__xx) * Fx__fl) + (ms * (i__xz * Fy__fl * Wf + 2 * i__zz * Tw__fl) * (h__Gs - z__static)) / 0.2e1) * delta__fl + ((((h__Gs - z__static) * (Lf * i__xz - Rf * i__zz + h__Gs * i__zz - i__zz * z__static) * ms - i__xz * is__xz + i__zz * is__xx) * Fx__fr) - (ms * (i__xz * Fy__fr * Wf - 2 * i__zz * Tw__fr) * (h__Gs - z__static)) / 0.2e1) * delta__fr - (ms * i__xz * Wf * (h__Gs - z__static) * Fx__fl) / 0.2e1 + (ms * i__xz * Wf * (h__Gs - z__static) * Fx__fr) / 0.2e1 + (((h__Gs - z__static) * (Lf * i__xz + h__Gs * i__zz - i__zz * z__static) * ms - i__xz * is__xz + i__zz * is__xx) * Fy__fl) + (((h__Gs - z__static) * (Lf * i__xz + h__Gs * i__zz - i__zz * z__static) * ms - i__xz * is__xz + i__zz * is__xx) * Fy__fr) + (((h__Gs - z__static) * (-Lr * i__xz + h__Gs * i__zz - i__zz * z__static) * ms - i__xz * is__xz + i__zz * is__xx) * Fy__rl) + (((h__Gs - z__static) * (-Lr * i__xz + h__Gs * i__zz - i__zz * z__static) * ms - i__xz * is__xz + i__zz * is__xx) * Fy__rr) + (h__Gs - z__static) * ((i__zz * Fz__fl * Wf) / 0.2e1 - (i__zz * Fz__fr * Wf) / 0.2e1 + (i__zz * Fz__rl * Wr) / 0.2e1 - (i__zz * Fz__rr * Wr) / 0.2e1 + i__xz * (-(Wr * Fx__rl) / 0.2e1 + (Wr * Fx__rr) / 0.2e1 + AM__fl + AM__fr + AM__rl + AM__rr)) * ms)) / (2 * (ms * (h__Gs - z__static) * (ms - m) * z - z__static * (h__Gs - z__static) * ms ^ 2 + m * z__static * (h__Gs - z__static) * ms - is__yy * m) * is__xz * (ms * (h__Gs - z__static) * (ms - m) * z - z__static * (h__Gs - z__static) * ms ^ 2 + m * z__static * (h__Gs - z__static) * ms - m * (is__xx + is__zz)) * mu + 2 * (h__Gs - z__static) ^ 2 * (ms * (h__Gs - z__static) * (ms - m) * z - z__static * (h__Gs - z__static) * ms ^ 2 + m * z__static * (h__Gs - z__static) * ms - is__xx * m) * is__zz * ms ^ 2 * phi ^ 2 + 2 * (ms * i__zz * (h__Gs - z__static) * (ms - m) * z - i__zz * z__static * (h__Gs - z__static) * ms ^ 2 + i__zz * m * z__static * (h__Gs - z__static) * ms + m * (i__xz * is__xz - i__zz * is__xx)) * (ms * (h__Gs - z__static) * (ms - m) * z - z__static * (h__Gs - z__static) * ms ^ 2 + m * z__static * (h__Gs - z__static) * ms - is__yy * m));
z_DDot       = (-m * g - FAz__f - FAz__r + Fz__fl + Fz__fr + Fz__rl + Fz__rr) / ms;
% 3 Euler equations
phi_DDot     = (-(2 * (h__Gs - z__static) * (ms * (h__Gs - z__static) * (ms - m) * z - z__static * (h__Gs - z__static) * ms ^ 2 + m * z__static * (h__Gs - z__static) * ms - m * (is__xx - is__zz)) * (((is__xx - is__yy - is__zz) * Omega ^ 2 + (h__Gs - z__static) * (-m * g + g * ms - FAz__f - FAz__r + Fz__fl + Fz__fr + Fz__rl + Fz__rr)) * (h__Gs - z__static) * ms * phi + (ms * (h__Gs - z__static) * (ms - m) * z - z__static * (h__Gs - z__static) * ms ^ 2 + m * z__static * (h__Gs - z__static) * ms - is__yy * m) * u * Omega) * ms * mu ^ 2) + ((-(2 * (h__Gs - z__static) ^ 2 * (ms - m) * (-2 * is__xz * (ms - m) * Omega ^ 2 + ms * v * (h__Gs - z__static) * (ms - m) * Omega - ms * (-delta__fl * Fy__fl - delta__fr * Fy__fr + Fx__fl + Fx__fr + Fx__rl + Fx__rr) * (h__Gs - z__static)) * ms ^ 2 * z ^ 2) - 0.4e1 * (h__Gs - z__static) * ((((h__Gs - z__static) * ((-i__xz + 4 * is__xz) * z__static + h__Gs * i__xz) * ms ^ 2) - (4 * is__xz * m * z__static * (h__Gs - z__static) * ms) + 0.4e1 * is__xz * (is__yy - is__zz / 0.2e1) * m) * (ms - m) * (Omega ^ 2) / 0.2e1 - (h__Gs - z__static) * (ms - m) * (-(ms * iwa__f * omega__fl * (h__Gs - z__static) * delta__fl) / 0.2e1 - (ms * iwa__f * omega__fr * (h__Gs - z__static) * delta__fr) / 0.2e1 + ((z__static * (h__Gs - z__static) * ms ^ 2) - (m * z__static * (h__Gs - z__static) * ms) + (m * (is__xx + is__yy - is__zz)) / 0.2e1) * v + (ms * phi__dot * (is__xx - is__yy - is__zz) * (h__Gs - z__static)) / 0.2e1) * ms * Omega + ((((h__Gs - z__static) * (h__Gs - 2 * z__static) * ms ^ 2 + (-(h__Gs - z__static) * (h__Gs - 2 * z__static) * m + is__yy) * ms - m * (is__xx + is__yy - is__zz)) * Fy__fl * ms * delta__fl) / 0.2e1 + (((h__Gs - z__static) * (h__Gs - 2 * z__static) * ms ^ 2 + (-(h__Gs - z__static) * (h__Gs - 2 * z__static) * m + is__yy) * ms - m * (is__xx + is__yy - is__zz)) * Fy__fr * ms * delta__fr) / 0.2e1 - (((h__Gs - z__static) * (h__Gs - 2 * z__static - Rf) * ms ^ 2 + (-(h__Gs - z__static) * (h__Gs - 2 * z__static - Rf) * m + is__yy) * ms - m * (is__xx + is__yy - is__zz)) * ms * Fx__fl) / 0.2e1 - (((h__Gs - z__static) * (h__Gs - 2 * z__static - Rf) * ms ^ 2 + (-(h__Gs - z__static) * (h__Gs - 2 * z__static - Rf) * m + is__yy) * ms - m * (is__xx + is__yy - is__zz)) * ms * Fx__fr) / 0.2e1 - (((h__Gs - z__static) * (h__Gs - 2 * z__static - Rr) * ms ^ 2 + (-(h__Gs - z__static) * (h__Gs - 2 * z__static - Rr) * m + is__yy) * ms - m * (is__xx + is__yy - is__zz)) * ms * Fx__rl) / 0.2e1 - (((h__Gs - z__static) * (h__Gs - 2 * z__static - Rr) * ms ^ 2 + (-(h__Gs - z__static) * (h__Gs - 2 * z__static - Rr) * m + is__yy) * ms - m * (is__xx + is__yy - is__zz)) * ms * Fx__rr) / 0.2e1 + (ms - m) * ((-(Lf * (h__Gs - z__static) * ms ^ 2) / 0.2e1 + (is__xz * m)) * Fz__fl + (-(Lf * (h__Gs - z__static) * ms ^ 2) / 0.2e1 + (is__xz * m)) * Fz__fr + ((Lr * (h__Gs - z__static) * ms ^ 2) / 0.2e1 + (is__xz * m)) * Fz__rl + ((Lr * (h__Gs - z__static) * ms ^ 2) / 0.2e1 + (is__xz * m)) * Fz__rr + ((Lf * (h__Gs - z__static) * ms ^ 2) / 0.2e1 - (is__xz * m)) * FAz__f + (-(Lr * (h__Gs - z__static) * ms ^ 2) / 0.2e1 - (is__xz * m)) * FAz__r + (((h__Gs - z__static) ^ 2 * ms + is__yy) * ms * FAxc) / 0.2e1 - (ms ^ 2 * (h__Gs - z__static) * Tw__fl) / 0.2e1 - (ms ^ 2 * (h__Gs - z__static) * Tw__fr) / 0.2e1 - (ms ^ 2 * (h__Gs - z__static) * Tw__rl) / 0.2e1 - (ms ^ 2 * (h__Gs - z__static) * Tw__rr) / 0.2e1 + (g * is__xz * m * (ms - m)))) * (h__Gs - z__static)) * ms * z + ((2 * ((-i__xz + 2 * is__xz) * z__static + h__Gs * i__xz) * (h__Gs - z__static) ^ 2 * z__static * ms ^ 4) - (2 * (h__Gs - z__static) ^ 2 * z__static * m * ((-i__xz + 4 * is__xz) * z__static + h__Gs * i__xz) * ms ^ 3) + 0.4e1 * ((is__xz * z__static ^ 2 * (h__Gs - z__static) * m) + (((i__xz - is__xz) * is__zz) + (i__xz / 0.2e1 + (2 * is__xz)) * is__yy - (i__xz * is__xx)) * z__static + i__xz * h__Gs * (is__xx - is__yy / 0.2e1 - is__zz)) * (h__Gs - z__static) * m * (ms ^ 2) - 0.8e1 * is__xz * (h__Gs - z__static) * z__static * (is__yy - is__zz / 0.2e1) * (m ^ 2) * ms + (4 * is__xz * is__yy * m ^ 2 * (is__yy - is__zz))) * (Omega ^ 2) - (2 * (h__Gs - z__static) * (-ms * iwa__f * omega__fl * (h__Gs - z__static) * delta__fl - ms * iwa__f * omega__fr * (h__Gs - z__static) * delta__fr + (z__static * (h__Gs - z__static) * ms ^ 2 - m * z__static * (h__Gs - z__static) * ms + is__yy * m) * v + ms * phi__dot * (is__xx - is__yy - is__zz) * (h__Gs - z__static)) * (z__static * (h__Gs - z__static) * ms ^ 2 - m * z__static * (h__Gs - z__static) * ms + m * (is__xx - is__zz)) * ms * Omega) + (2 * (h__Gs - z__static) * (((h__Gs - z__static) ^ 2 * ms + is__yy) * Fy__fl * (z__static * (h__Gs - z__static) * ms ^ 2 - m * z__static * (h__Gs - z__static) * ms + m * (is__xx - is__zz)) * ms * delta__fl + ((h__Gs - z__static) ^ 2 * ms + is__yy) * Fy__fr * (z__static * (h__Gs - z__static) * ms ^ 2 - m * z__static * (h__Gs - z__static) * ms + m * (is__xx - is__zz)) * ms * delta__fr - ((h__Gs - z__static) * (h__Gs - z__static - Rf) * ms + is__yy) * (z__static * (h__Gs - z__static) * ms ^ 2 - m * z__static * (h__Gs - z__static) * ms + m * (is__xx - is__zz)) * ms * Fx__fl - ((h__Gs - z__static) * (h__Gs - z__static - Rf) * ms + is__yy) * (z__static * (h__Gs - z__static) * ms ^ 2 - m * z__static * (h__Gs - z__static) * ms + m * (is__xx - is__zz)) * ms * Fx__fr - ((h__Gs - z__static) * (h__Gs - z__static - Rr) * ms + is__yy) * (z__static * (h__Gs - z__static) * ms ^ 2 - m * z__static * (h__Gs - z__static) * ms + m * (is__xx - is__zz)) * ms * Fx__rl - ((h__Gs - z__static) * (h__Gs - z__static - Rr) * ms + is__yy) * (z__static * (h__Gs - z__static) * ms ^ 2 - m * z__static * (h__Gs - z__static) * ms + m * (is__xx - is__zz)) * ms * Fx__rr + (-z__static * Lf * (h__Gs - z__static) ^ 2 * ms ^ 4 + m * z__static * Lf * (h__Gs - z__static) ^ 2 * ms ^ 3 + (h__Gs - z__static) * ((-i__xz + 2 * is__xz) * z__static + h__Gs * i__xz - Lf * (is__xx - is__zz)) * m * ms ^ 2 - 2 * is__xz * m ^ 2 * z__static * (h__Gs - z__static) * ms + 2 * is__xz * is__yy * m ^ 2) * Fz__fl + (-z__static * Lf * (h__Gs - z__static) ^ 2 * ms ^ 4 + m * z__static * Lf * (h__Gs - z__static) ^ 2 * ms ^ 3 + (h__Gs - z__static) * ((-i__xz + 2 * is__xz) * z__static + h__Gs * i__xz - Lf * (is__xx - is__zz)) * m * ms ^ 2 - 2 * is__xz * m ^ 2 * z__static * (h__Gs - z__static) * ms + 2 * is__xz * is__yy * m ^ 2) * Fz__fr + (Lr * z__static * (h__Gs - z__static) ^ 2 * ms ^ 4 - m * z__static * Lr * (h__Gs - z__static) ^ 2 * ms ^ 3 + (h__Gs - z__static) * ((-i__xz + 2 * is__xz) * z__static + h__Gs * i__xz + Lr * (is__xx - is__zz)) * m * ms ^ 2 - 2 * is__xz * m ^ 2 * z__static * (h__Gs - z__static) * ms + 2 * is__xz * is__yy * m ^ 2) * Fz__rl + (Lr * z__static * (h__Gs - z__static) ^ 2 * ms ^ 4 - m * z__static * Lr * (h__Gs - z__static) ^ 2 * ms ^ 3 + (h__Gs - z__static) * ((-i__xz + 2 * is__xz) * z__static + h__Gs * i__xz + Lr * (is__xx - is__zz)) * m * ms ^ 2 - 2 * is__xz * m ^ 2 * z__static * (h__Gs - z__static) * ms + 2 * is__xz * is__yy * m ^ 2) * Fz__rr + (z__static * Lf * (h__Gs - z__static) ^ 2 * ms ^ 4 - m * z__static * Lf * (h__Gs - z__static) ^ 2 * ms ^ 3 - (h__Gs - z__static) * ((-i__xz + 2 * is__xz) * z__static + h__Gs * i__xz - Lf * (is__xx - is__zz)) * m * ms ^ 2 + 2 * is__xz * m ^ 2 * z__static * (h__Gs - z__static) * ms - 2 * is__xz * is__yy * m ^ 2) * FAz__f + (-Lr * z__static * (h__Gs - z__static) ^ 2 * ms ^ 4 + m * z__static * Lr * (h__Gs - z__static) ^ 2 * ms ^ 3 - (h__Gs - z__static) * ((-i__xz + 2 * is__xz) * z__static + h__Gs * i__xz + Lr * (is__xx - is__zz)) * m * ms ^ 2 + 2 * is__xz * m ^ 2 * z__static * (h__Gs - z__static) * ms - 2 * is__xz * is__yy * m ^ 2) * FAz__r + ((h__Gs - z__static) ^ 2 * ms + is__yy) * (z__static * (h__Gs - z__static) * ms ^ 2 - m * z__static * (h__Gs - z__static) * ms + m * (is__xx - is__zz)) * ms * FAxc - (h__Gs - z__static) * (z__static * (h__Gs - z__static) * ms ^ 2 - m * z__static * (h__Gs - z__static) * ms + m * (is__xx - is__zz)) * ms ^ 2 * Tw__fl - (h__Gs - z__static) * (z__static * (h__Gs - z__static) * ms ^ 2 - m * z__static * (h__Gs - z__static) * ms + m * (is__xx - is__zz)) * ms ^ 2 * Tw__fr - (h__Gs - z__static) * (z__static * (h__Gs - z__static) * ms ^ 2 - m * z__static * (h__Gs - z__static) * ms + m * (is__xx - is__zz)) * ms ^ 2 * Tw__rl - (h__Gs - z__static) * (z__static * (h__Gs - z__static) * ms ^ 2 - m * z__static * (h__Gs - z__static) * ms + m * (is__xx - is__zz)) * ms ^ 2 * Tw__rr + (ms - m) * m * g * (((-i__xz + 2 * is__xz) * z__static + h__Gs * i__xz) * (h__Gs - z__static) * ms ^ 2 - 2 * is__xz * m * z__static * (h__Gs - z__static) * ms + 2 * is__xz * is__yy * m)))) * phi + 0.4e1 * (ms * (h__Gs - z__static) * (ms - m) * z - z__static * (h__Gs - z__static) * ms ^ 2 + m * z__static * (h__Gs - z__static) * ms - is__yy * m) * (((is__xz * mu__dot * (h__Gs - z__static) * (ms - m) * Omega) + (((Lf * (h__Gs - z__static) * ms) / 0.2e1 - (Lf * (h__Gs - z__static) * m) / 0.2e1 - is__xz) * Fx__fl + (Fy__fl * Wf * (h__Gs - z__static) * (ms - m)) / 0.4e1) * delta__fl + (((Lf * (h__Gs - z__static) * ms) / 0.2e1 - (Lf * (h__Gs - z__static) * m) / 0.2e1 - is__xz) * Fx__fr - (Fy__fr * Wf * (h__Gs - z__static) * (ms - m)) / 0.4e1) * delta__fr - (Wf * (h__Gs - z__static) * (ms - m) * Fx__fl) / 0.4e1 + (Wf * (h__Gs - z__static) * (ms - m) * Fx__fr) / 0.4e1 + ((Lf * (h__Gs - z__static) * ms) / 0.2e1 - (Lf * (h__Gs - z__static) * m) / 0.2e1 - is__xz) * Fy__fl + ((Lf * (h__Gs - z__static) * ms) / 0.2e1 - (Lf * (h__Gs - z__static) * m) / 0.2e1 - is__xz) * Fy__fr - (Wr * (h__Gs - z__static) * (ms - m) * Fx__rl) / 0.4e1 + (Wr * (h__Gs - z__static) * (ms - m) * Fx__rr) / 0.4e1 + (-(Lr * (h__Gs - z__static) * ms) / 0.2e1 + (Lr * (h__Gs - z__static) * m) / 0.2e1 - is__xz) * Fy__rl + (-(Lr * (h__Gs - z__static) * ms) / 0.2e1 + (Lr * (h__Gs - z__static) * m) / 0.2e1 - is__xz) * Fy__rr + ((AM__fl + AM__fr + AM__rl + AM__rr) * (h__Gs - z__static) * (ms - m)) / 0.2e1) * ms * z + (-(is__xz * (z__static * (h__Gs - z__static) * ms ^ 2 - m * z__static * (h__Gs - z__static) * ms + is__yy * m) * mu__dot) + ((ms * i__xz * (h__Gs - z__static) * u - 2 * is__xz * (iwa__f * omega__fl + iwa__f * omega__fr + iwa__r * (omega__rl + omega__rr))) * m) / 0.2e1) * Omega + ((-(z__static * Lf * (h__Gs - z__static) * ms ^ 2) / 0.2e1 + (z__static * (Lf * (h__Gs - z__static) * m + 2 * is__xz) * ms) / 0.2e1 - m * ((h__Gs * is__xz) + (is__xx * Lf) / 0.2e1 - (is__xz * Rf) - (is__zz * Lf) / 0.2e1)) * Fx__fl - (Wf * (z__static * (h__Gs - z__static) * ms ^ 2 - m * z__static * (h__Gs - z__static) * ms + m * (is__xx - is__zz)) * Fy__fl) / 0.4e1 - (is__xz * m * Tw__fl)) * delta__fl + ((-(z__static * Lf * (h__Gs - z__static) * ms ^ 2) / 0.2e1 + (z__static * (Lf * (h__Gs - z__static) * m + 2 * is__xz) * ms) / 0.2e1 - m * ((h__Gs * is__xz) + (is__xx * Lf) / 0.2e1 - (is__xz * Rf) - (is__zz * Lf) / 0.2e1)) * Fx__fr + (Wf * (z__static * (h__Gs - z__static) * ms ^ 2 - m * z__static * (h__Gs - z__static) * ms + m * (is__xx - is__zz)) * Fy__fr) / 0.4e1 - (is__xz * m * Tw__fr)) * delta__fr + (Wf * (z__static * (h__Gs - z__static) * ms ^ 2 - m * z__static * (h__Gs - z__static) * ms + m * (is__xx - is__zz)) * Fx__fl) / 0.4e1 - (Wf * (z__static * (h__Gs - z__static) * ms ^ 2 - m * z__static * (h__Gs - z__static) * ms + m * (is__xx - is__zz)) * Fx__fr) / 0.4e1 + (-(z__static * Lf * (h__Gs - z__static) * ms ^ 2) / 0.2e1 + (z__static * (Lf * (h__Gs - z__static) * m + 2 * is__xz) * ms) / 0.2e1 - m * ((h__Gs * is__xz) + (Lf * (is__xx - is__zz)) / 0.2e1)) * Fy__fl + (-(z__static * Lf * (h__Gs - z__static) * ms ^ 2) / 0.2e1 + (z__static * (Lf * (h__Gs - z__static) * m + 2 * is__xz) * ms) / 0.2e1 - m * ((h__Gs * is__xz) + (Lf * (is__xx - is__zz)) / 0.2e1)) * Fy__fr + (Wr * (z__static * (h__Gs - z__static) * ms ^ 2 - m * z__static * (h__Gs - z__static) * ms + m * (is__xx - is__zz)) * Fx__rl) / 0.4e1 - (Wr * (z__static * (h__Gs - z__static) * ms ^ 2 - m * z__static * (h__Gs - z__static) * ms + m * (is__xx - is__zz)) * Fx__rr) / 0.4e1 + ((Lr * z__static * (h__Gs - z__static) * ms ^ 2) / 0.2e1 - (z__static * (Lr * (h__Gs - z__static) * m - 2 * is__xz) * ms) / 0.2e1 - ((h__Gs * is__xz) - (Lr * (is__xx - is__zz)) / 0.2e1) * m) * Fy__rl + ((Lr * z__static * (h__Gs - z__static) * ms ^ 2) / 0.2e1 - (z__static * (Lr * (h__Gs - z__static) * m - 2 * is__xz) * ms) / 0.2e1 - ((h__Gs * is__xz) - (Lr * (is__xx - is__zz)) / 0.2e1) * m) * Fy__rr - (is__xz * m * Fz__fl * Wf) / 0.2e1 + (is__xz * m * Fz__fr * Wf) / 0.2e1 - (is__xz * m * Fz__rl * Wr) / 0.2e1 + (is__xz * m * Fz__rr * Wr) / 0.2e1 - ((z__static * (h__Gs - z__static) * ms ^ 2 - m * z__static * (h__Gs - z__static) * ms + m * (is__xx - is__zz)) * (AM__fl + AM__fr + AM__rl + AM__rr)) / 0.2e1)) * mu - (2 * (h__Gs - z__static) ^ 2 * (-ms * Omega ^ 2 * (h__Gs - z__static) * (ms - m) * z + (z__static * (h__Gs - z__static) * ms ^ 2 - m * z__static * (h__Gs - z__static) * ms + m * (is__yy - is__zz)) * Omega ^ 2 + m * (h__Gs - z__static) * (-m * g + g * ms - FAz__f - FAz__r + Fz__fl + Fz__fr + Fz__rl + Fz__rr)) * is__zz * ms ^ 2 * phi ^ 3) + 0.4e1 * ((h__Gs - z__static) ^ 2) * is__zz * (((mu__dot * (h__Gs - z__static) * (ms - m) * Omega) - (Fx__fr * delta__fr) / 0.2e1 - (Fx__fl * delta__fl) / 0.2e1 - Fy__rr / 0.2e1 - Fy__rl / 0.2e1 - Fy__fr / 0.2e1 - Fy__fl / 0.2e1) * ms * z + ((-(z__static * (h__Gs - z__static) * ms ^ 2) + (m * z__static * (h__Gs - z__static) * ms) - (m * (is__xx + is__yy - is__zz)) / 0.2e1) * mu__dot - ((iwa__f * omega__fl + iwa__f * omega__fr + iwa__r * (omega__rl + omega__rr)) * m) / 0.2e1) * Omega + (((z__static * ms) / 0.2e1 - (m * (h__Gs - Rf)) / 0.2e1) * Fx__fl - (m * Tw__fl) / 0.2e1) * delta__fl + (((z__static * ms) / 0.2e1 - (m * (h__Gs - Rf)) / 0.2e1) * Fx__fr - (m * Tw__fr) / 0.2e1) * delta__fr + ((z__static * ms) / 0.2e1 - (m * h__Gs) / 0.2e1) * Fy__fl + ((z__static * ms) / 0.2e1 - (m * h__Gs) / 0.2e1) * Fy__fr + ((z__static * ms) / 0.2e1 - (m * h__Gs) / 0.2e1) * Fy__rl + ((z__static * ms) / 0.2e1 - (m * h__Gs) / 0.2e1) * Fy__rr - ((Wf * Fz__fl - Wf * Fz__fr + Wr * (Fz__rl - Fz__rr)) * m) / 0.4e1) * (ms ^ 2) * (phi ^ 2) + ((2 * ms ^ 2 * i__zz * Omega ^ 2 * (h__Gs - z__static) ^ 2 * (ms - m) ^ 2 * z ^ 2) - 0.2e1 * (h__Gs - z__static) * (0.2e1 * ((z__static * (h__Gs - z__static) * ms ^ 2) - (m * z__static * (h__Gs - z__static) * ms) + m * (is__yy - is__zz / 0.2e1)) * (ms - m) * i__zz * (Omega ^ 2) - (ms * i__xz * m * v * (h__Gs - z__static) * (ms - m) * Omega) + ((h__Gs - z__static) * (-ms * i__xz * Fy__fl * delta__fl - ms * i__xz * Fy__fr * delta__fr + ms * i__xz * Fx__fl + ms * i__xz * Fx__fr + ms * i__xz * Fx__rl + ms * i__xz * Fx__rr + i__zz * (ms - m) * (-m * g + g * ms - FAz__f - FAz__r + Fz__fl + Fz__fr + Fz__rl + Fz__rr)) * m)) * ms * z + ((2 * i__zz * z__static ^ 2 * (h__Gs - z__static) ^ 2 * ms ^ 4) - (4 * i__zz * m * z__static ^ 2 * (h__Gs - z__static) ^ 2 * ms ^ 3) + (2 * (h__Gs - z__static) * (i__zz * z__static ^ 2 * (h__Gs - z__static) * m + (-i__xz ^ 2 + 2 * i__zz * is__yy - i__zz * is__zz) * z__static + i__xz ^ 2 * h__Gs) * m * ms ^ 2) - 0.4e1 * (h__Gs - z__static) * z__static * i__zz * (m ^ 2) * (is__yy - is__zz / 0.2e1) * ms + (2 * i__zz * is__yy * m ^ 2 * (is__yy - is__zz))) * (Omega ^ 2) - (2 * i__xz * (h__Gs - z__static) * (-ms * iwa__f * omega__fl * (h__Gs - z__static) * delta__fl - ms * iwa__f * omega__fr * (h__Gs - z__static) * delta__fr + (z__static * (h__Gs - z__static) * ms ^ 2 - m * z__static * (h__Gs - z__static) * ms + is__yy * m) * v + ms * phi__dot * (is__xx - is__yy - is__zz) * (h__Gs - z__static)) * m * ms * Omega) + (2 * (((h__Gs - z__static) ^ 2 * ms + is__yy) * i__xz * Fy__fl * ms * delta__fl + ((h__Gs - z__static) ^ 2 * ms + is__yy) * i__xz * Fy__fr * ms * delta__fr - ((h__Gs - z__static) * (h__Gs - z__static - Rf) * ms + is__yy) * i__xz * ms * Fx__fl - ((h__Gs - z__static) * (h__Gs - z__static - Rf) * ms + is__yy) * i__xz * ms * Fx__fr + (-(Lf * i__xz - i__zz * z__static) * (h__Gs - z__static) * ms ^ 2 - i__zz * m * z__static * (h__Gs - z__static) * ms + i__zz * is__yy * m) * Fz__fl + (-(Lf * i__xz - i__zz * z__static) * (h__Gs - z__static) * ms ^ 2 - i__zz * m * z__static * (h__Gs - z__static) * ms + i__zz * is__yy * m) * Fz__fr + ((Lr * i__xz + i__zz * z__static) * (h__Gs - z__static) * ms ^ 2 - i__zz * m * z__static * (h__Gs - z__static) * ms + i__zz * is__yy * m) * Fz__rl + ((Lr * i__xz + i__zz * z__static) * (h__Gs - z__static) * ms ^ 2 - i__zz * m * z__static * (h__Gs - z__static) * ms + i__zz * is__yy * m) * Fz__rr + ((Lf * i__xz - i__zz * z__static) * (h__Gs - z__static) * ms ^ 2 + i__zz * m * z__static * (h__Gs - z__static) * ms - i__zz * is__yy * m) * FAz__f + (-(Lr * i__xz + i__zz * z__static) * (h__Gs - z__static) * ms ^ 2 + i__zz * m * z__static * (h__Gs - z__static) * ms - i__zz * is__yy * m) * FAz__r - i__xz * ((h__Gs - z__static) * (h__Gs - z__static - Rr) * ms + is__yy) * ms * Fx__rl - i__xz * ((h__Gs - z__static) * (h__Gs - z__static - Rr) * ms + is__yy) * ms * Fx__rr - ms ^ 2 * i__xz * (h__Gs - z__static) * Tw__fl - ms ^ 2 * i__xz * (h__Gs - z__static) * Tw__fr + ((h__Gs - z__static) ^ 2 * ms + is__yy) * i__xz * ms * FAxc - ms ^ 2 * i__xz * (h__Gs - z__static) * Tw__rl - ms ^ 2 * i__xz * (h__Gs - z__static) * Tw__rr + (ms - m) * i__zz * (z__static * (h__Gs - z__static) * ms ^ 2 - m * z__static * (h__Gs - z__static) * ms + is__yy * m) * g) * (h__Gs - z__static) * m)) * phi + 0.4e1 * (ms * (h__Gs - z__static) * (ms - m) * z - z__static * (h__Gs - z__static) * ms ^ 2 + m * z__static * (h__Gs - z__static) * ms - is__yy * m) * (((mu__dot * (h__Gs - z__static) * (ms - m) * Omega) - (Fx__fr * delta__fr) / 0.2e1 - (Fx__fl * delta__fl) / 0.2e1 - Fy__rr / 0.2e1 - Fy__rl / 0.2e1 - Fy__fr / 0.2e1 - Fy__fl / 0.2e1) * i__zz * ms * z + ((-(i__zz * z__static * (h__Gs - z__static) * ms ^ 2) + (i__zz * m * z__static * (h__Gs - z__static) * ms) + m * ((i__xz * is__xz) - (i__zz * is__xx) / 0.2e1 - (i__zz * is__yy) / 0.2e1 + (i__zz * is__zz) / 0.2e1)) * mu__dot - ((iwa__f * omega__fl + iwa__f * omega__fr + iwa__r * (omega__rl + omega__rr)) * i__zz * m) / 0.2e1) * Omega + (((ms * i__zz * z__static) / 0.2e1 - (m * (Lf * i__xz - Rf * i__zz + h__Gs * i__zz)) / 0.2e1) * Fx__fl - (m * (i__xz * Fy__fl * Wf + 2 * i__zz * Tw__fl)) / 0.4e1) * delta__fl + (((ms * i__zz * z__static) / 0.2e1 - (m * (Lf * i__xz - Rf * i__zz + h__Gs * i__zz)) / 0.2e1) * Fx__fr + (m * (i__xz * Fy__fr * Wf - 2 * i__zz * Tw__fr)) / 0.4e1) * delta__fr + (i__xz * m * Fx__fl * Wf) / 0.4e1 - (i__xz * m * Fx__fr * Wf) / 0.4e1 + ((ms * i__zz * z__static) / 0.2e1 - (m * (Lf * i__xz + h__Gs * i__zz)) / 0.2e1) * Fy__fl + ((ms * i__zz * z__static) / 0.2e1 - (m * (Lf * i__xz + h__Gs * i__zz)) / 0.2e1) * Fy__fr + (i__xz * m * Fx__rl * Wr) / 0.4e1 - (i__xz * m * Fx__rr * Wr) / 0.4e1 + ((ms * i__zz * z__static) / 0.2e1 - (m * (-Lr * i__xz + h__Gs * i__zz)) / 0.2e1) * Fy__rl + ((ms * i__zz * z__static) / 0.2e1 - (m * (-Lr * i__xz + h__Gs * i__zz)) / 0.2e1) * Fy__rr - ((i__zz * Fz__fl * Wf) / 0.2e1 - (i__zz * Fz__fr * Wf) / 0.2e1 + (i__zz * Fz__rl * Wr) / 0.2e1 - (i__zz * Fz__rr * Wr) / 0.2e1 + (i__xz * (AM__fl + AM__fr + AM__rl + AM__rr))) * m / 0.2e1)) / (2 * (ms * (h__Gs - z__static) * (ms - m) * z - z__static * (h__Gs - z__static) * ms ^ 2 + m * z__static * (h__Gs - z__static) * ms - is__yy * m) * is__xz * (ms * (h__Gs - z__static) * (ms - m) * z - z__static * (h__Gs - z__static) * ms ^ 2 + m * z__static * (h__Gs - z__static) * ms - m * (is__xx + is__zz)) * mu + 2 * (h__Gs - z__static) ^ 2 * (ms * (h__Gs - z__static) * (ms - m) * z - z__static * (h__Gs - z__static) * ms ^ 2 + m * z__static * (h__Gs - z__static) * ms - is__xx * m) * is__zz * ms ^ 2 * phi ^ 2 + 2 * (ms * i__zz * (h__Gs - z__static) * (ms - m) * z - i__zz * z__static * (h__Gs - z__static) * ms ^ 2 + i__zz * m * z__static * (h__Gs - z__static) * ms + m * (i__xz * is__xz - i__zz * is__xx)) * (ms * (h__Gs - z__static) * (ms - m) * z - z__static * (h__Gs - z__static) * ms ^ 2 + m * z__static * (h__Gs - z__static) * ms - is__yy * m));
mu_DDot      = (((2 * (h__Gs - z__static) ^ 2 * (ms - m) * (-is__xz * (ms - m) * Omega ^ 2 + ms * v * (h__Gs - z__static) * (ms - m) * Omega - ms * (-delta__fl * Fy__fl - delta__fr * Fy__fr + Fx__fl + Fx__fr + Fx__rl + Fx__rr) * (h__Gs - z__static)) * ms ^ 2 * z ^ 2) + 0.2e1 * (h__Gs - z__static) * (((h__Gs - z__static) ^ 2 * (ms - m) * ((is__xx - is__yy) * Omega ^ 2 + (h__Gs - z__static) * (-m * g + g * ms - FAz__f - FAz__r + Fz__fl + Fz__fr + Fz__rl + Fz__rr)) * ms ^ 2 * mu) + ((((-i__xz + 2 * is__xz) * z__static + h__Gs * i__xz) * (h__Gs - z__static) * ms ^ 2 - 2 * is__xz * m * z__static * (h__Gs - z__static) * ms + 2 * is__xz * m * (is__yy - is__zz)) * (ms - m) * Omega ^ 2) - 0.2e1 * (h__Gs - z__static) * (-(ms * iwa__f * omega__fl * (h__Gs - z__static) * delta__fl) / 0.2e1 - (ms * iwa__f * omega__fr * (h__Gs - z__static) * delta__fr) / 0.2e1 + (ms * (is__xx - is__yy + is__zz) * (h__Gs - z__static) * phi__dot) / 0.2e1 + ((z__static * (h__Gs - z__static) * ms ^ 2) - (m * z__static * (h__Gs - z__static) * ms) + (m * (is__xx + is__yy - is__zz)) / 0.2e1) * v) * (ms - m) * ms * Omega + ((h__Gs - z__static) * (Fy__fl * ((h__Gs - z__static) * (h__Gs - 2 * z__static) * ms ^ 2 + (-(h__Gs - z__static) * (h__Gs - 2 * z__static) * m + is__yy - is__zz) * ms - m * (is__xx + is__yy - is__zz)) * ms * delta__fl + Fy__fr * ((h__Gs - z__static) * (h__Gs - 2 * z__static) * ms ^ 2 + (-(h__Gs - z__static) * (h__Gs - 2 * z__static) * m + is__yy - is__zz) * ms - m * (is__xx + is__yy - is__zz)) * ms * delta__fr - ((h__Gs - z__static) * (h__Gs - 2 * z__static - Rf) * ms ^ 2 + (-(h__Gs - z__static) * (h__Gs - 2 * z__static - Rf) * m + is__yy - is__zz) * ms - m * (is__xx + is__yy - is__zz)) * ms * Fx__fl - ((h__Gs - z__static) * (h__Gs - 2 * z__static - Rf) * ms ^ 2 + (-(h__Gs - z__static) * (h__Gs - 2 * z__static - Rf) * m + is__yy - is__zz) * ms - m * (is__xx + is__yy - is__zz)) * ms * Fx__fr - ((h__Gs - z__static) * (h__Gs - 2 * z__static - Rr) * ms ^ 2 + (-(h__Gs - z__static) * (h__Gs - 2 * z__static - Rr) * m + is__yy - is__zz) * ms - m * (is__xx + is__yy - is__zz)) * ms * Fx__rl - ((h__Gs - z__static) * (h__Gs - 2 * z__static - Rr) * ms ^ 2 + (-(h__Gs - z__static) * (h__Gs - 2 * z__static - Rr) * m + is__yy - is__zz) * ms - m * (is__xx + is__yy - is__zz)) * ms * Fx__rr + ((-Lf * (h__Gs - z__static) * ms ^ 2 + is__xz * m) * Fz__fl + (-Lf * (h__Gs - z__static) * ms ^ 2 + is__xz * m) * Fz__fr + (Lr * (h__Gs - z__static) * ms ^ 2 + is__xz * m) * Fz__rl + (Lr * (h__Gs - z__static) * ms ^ 2 + is__xz * m) * Fz__rr + (Lf * (h__Gs - z__static) * ms ^ 2 - is__xz * m) * FAz__f + (-Lr * (h__Gs - z__static) * ms ^ 2 - is__xz * m) * FAz__r + ((h__Gs - z__static) ^ 2 * ms + is__yy - is__zz) * ms * FAxc - ms ^ 2 * (h__Gs - z__static) * Tw__fl - ms ^ 2 * (h__Gs - z__static) * Tw__fr - ms ^ 2 * (h__Gs - z__static) * Tw__rl - ms ^ 2 * (h__Gs - z__static) * Tw__rr + g * is__xz * m * (ms - m)) * (ms - m)))) * ms * z - (2 * (h__Gs - z__static) ^ 2 * ((is__xx - is__yy) * Omega ^ 2 + (h__Gs - z__static) * (-m * g + g * ms - FAz__f - FAz__r + Fz__fl + Fz__fr + Fz__rl + Fz__rr)) * (z__static * (h__Gs - z__static) * ms ^ 2 - m * z__static * (h__Gs - z__static) * ms + is__xx * m) * ms ^ 2 * mu) + ((-2 * (h__Gs - z__static) ^ 2 * z__static * ((-i__xz + is__xz) * z__static + h__Gs * i__xz) * ms ^ 4 + 2 * ((-i__xz + 2 * is__xz) * z__static + h__Gs * i__xz) * (h__Gs - z__static) ^ 2 * z__static * m * ms ^ 3 - 2 * (is__xz * z__static ^ 2 * (h__Gs - z__static) * m + ((2 * is__yy - 2 * is__zz) * is__xz - i__xz * is__xx) * z__static + h__Gs * i__xz * is__xx) * (h__Gs - z__static) * m * ms ^ 2 + 4 * is__xz * m ^ 2 * z__static * (is__yy - is__zz) * (h__Gs - z__static) * ms - 2 * is__xz * m ^ 2 * (is__yy - is__zz) ^ 2) * Omega ^ 2) + (2 * (h__Gs - z__static) * (-ms * iwa__f * omega__fl * (h__Gs - z__static) * delta__fl - ms * iwa__f * omega__fr * (h__Gs - z__static) * delta__fr + ms * (is__xx - is__yy + is__zz) * (h__Gs - z__static) * phi__dot + (z__static * (h__Gs - z__static) * ms ^ 2 - m * z__static * (h__Gs - z__static) * ms + m * (is__yy - is__zz)) * v) * (z__static * (h__Gs - z__static) * ms ^ 2 - m * z__static * (h__Gs - z__static) * ms + is__xx * m) * ms * Omega) - (2 * (h__Gs - z__static) * (((h__Gs - z__static) ^ 2 * ms + is__yy - is__zz) * Fy__fl * (z__static * (h__Gs - z__static) * ms ^ 2 - m * z__static * (h__Gs - z__static) * ms + is__xx * m) * ms * delta__fl + ((h__Gs - z__static) ^ 2 * ms + is__yy - is__zz) * Fy__fr * (z__static * (h__Gs - z__static) * ms ^ 2 - m * z__static * (h__Gs - z__static) * ms + is__xx * m) * ms * delta__fr - ((h__Gs - z__static) * (h__Gs - z__static - Rf) * ms + is__yy - is__zz) * (z__static * (h__Gs - z__static) * ms ^ 2 - m * z__static * (h__Gs - z__static) * ms + is__xx * m) * ms * Fx__fl - ((h__Gs - z__static) * (h__Gs - z__static - Rf) * ms + is__yy - is__zz) * (z__static * (h__Gs - z__static) * ms ^ 2 - m * z__static * (h__Gs - z__static) * ms + is__xx * m) * ms * Fx__fr - (z__static * (h__Gs - z__static) * ms ^ 2 - m * z__static * (h__Gs - z__static) * ms + is__xx * m) * ms * ((h__Gs - z__static) * (h__Gs - z__static - Rr) * ms + is__yy - is__zz) * Fx__rl - (z__static * (h__Gs - z__static) * ms ^ 2 - m * z__static * (h__Gs - z__static) * ms + is__xx * m) * ms * ((h__Gs - z__static) * (h__Gs - z__static - Rr) * ms + is__yy - is__zz) * Fx__rr + (-z__static * Lf * (h__Gs - z__static) ^ 2 * ms ^ 4 + m * z__static * Lf * (h__Gs - z__static) ^ 2 * ms ^ 3 - m * (is__xx * Lf - is__xz * z__static) * (h__Gs - z__static) * ms ^ 2 - is__xz * m ^ 2 * z__static * (h__Gs - z__static) * ms + is__xz * m ^ 2 * (is__yy - is__zz)) * Fz__fl + (-z__static * Lf * (h__Gs - z__static) ^ 2 * ms ^ 4 + m * z__static * Lf * (h__Gs - z__static) ^ 2 * ms ^ 3 - m * (is__xx * Lf - is__xz * z__static) * (h__Gs - z__static) * ms ^ 2 - is__xz * m ^ 2 * z__static * (h__Gs - z__static) * ms + is__xz * m ^ 2 * (is__yy - is__zz)) * Fz__fr + (Lr * z__static * (h__Gs - z__static) ^ 2 * ms ^ 4 - m * z__static * Lr * (h__Gs - z__static) ^ 2 * ms ^ 3 + m * (Lr * is__xx + is__xz * z__static) * (h__Gs - z__static) * ms ^ 2 - is__xz * m ^ 2 * z__static * (h__Gs - z__static) * ms + is__xz * m ^ 2 * (is__yy - is__zz)) * Fz__rl + (Lr * z__static * (h__Gs - z__static) ^ 2 * ms ^ 4 - m * z__static * Lr * (h__Gs - z__static) ^ 2 * ms ^ 3 + m * (Lr * is__xx + is__xz * z__static) * (h__Gs - z__static) * ms ^ 2 - is__xz * m ^ 2 * z__static * (h__Gs - z__static) * ms + is__xz * m ^ 2 * (is__yy - is__zz)) * Fz__rr + (z__static * Lf * (h__Gs - z__static) ^ 2 * ms ^ 4 - m * z__static * Lf * (h__Gs - z__static) ^ 2 * ms ^ 3 + m * (is__xx * Lf - is__xz * z__static) * (h__Gs - z__static) * ms ^ 2 + is__xz * m ^ 2 * z__static * (h__Gs - z__static) * ms - is__xz * m ^ 2 * (is__yy - is__zz)) * FAz__f + (-Lr * z__static * (h__Gs - z__static) ^ 2 * ms ^ 4 + m * z__static * Lr * (h__Gs - z__static) ^ 2 * ms ^ 3 - m * (Lr * is__xx + is__xz * z__static) * (h__Gs - z__static) * ms ^ 2 + is__xz * m ^ 2 * z__static * (h__Gs - z__static) * ms - is__xz * m ^ 2 * (is__yy - is__zz)) * FAz__r + ((h__Gs - z__static) ^ 2 * ms + is__yy - is__zz) * (z__static * (h__Gs - z__static) * ms ^ 2 - m * z__static * (h__Gs - z__static) * ms + is__xx * m) * ms * FAxc - (h__Gs - z__static) * (z__static * (h__Gs - z__static) * ms ^ 2 - m * z__static * (h__Gs - z__static) * ms + is__xx * m) * ms ^ 2 * Tw__fl - (h__Gs - z__static) * (z__static * (h__Gs - z__static) * ms ^ 2 - m * z__static * (h__Gs - z__static) * ms + is__xx * m) * ms ^ 2 * Tw__fr - (h__Gs - z__static) * (z__static * (h__Gs - z__static) * ms ^ 2 - m * z__static * (h__Gs - z__static) * ms + is__xx * m) * ms ^ 2 * Tw__rl - (h__Gs - z__static) * (z__static * (h__Gs - z__static) * ms ^ 2 - m * z__static * (h__Gs - z__static) * ms + is__xx * m) * ms ^ 2 * Tw__rr + is__xz * (z__static * (h__Gs - z__static) * ms ^ 2 - m * z__static * (h__Gs - z__static) * ms + m * (is__yy - is__zz)) * (ms - m) * m * g))) * phi ^ 2 + 0.2e1 * (((ms * u * mu * (h__Gs - z__static) ^ 2 * (ms - m) * Omega) + (((-Lf * (h__Gs - z__static) * ms + Lf * (h__Gs - z__static) * m + is__xz) * Fx__fl) - (Fy__fl * Wf * (h__Gs - z__static) * (ms - m)) / 0.2e1) * delta__fl + (((-Lf * (h__Gs - z__static) * ms + Lf * (h__Gs - z__static) * m + is__xz) * Fx__fr) + (Fy__fr * Wf * (h__Gs - z__static) * (ms - m)) / 0.2e1) * delta__fr + (Wf * (h__Gs - z__static) * (ms - m) * Fx__fl) / 0.2e1 - (Wf * (h__Gs - z__static) * (ms - m) * Fx__fr) / 0.2e1 + ((-Lf * (h__Gs - z__static) * ms + Lf * (h__Gs - z__static) * m + is__xz) * Fy__fl) + ((-Lf * (h__Gs - z__static) * ms + Lf * (h__Gs - z__static) * m + is__xz) * Fy__fr) + (Wr * (h__Gs - z__static) * (ms - m) * Fx__rl) / 0.2e1 - (Wr * (h__Gs - z__static) * (ms - m) * Fx__rr) / 0.2e1 + ((Lr * (h__Gs - z__static) * ms - Lr * (h__Gs - z__static) * m + is__xz) * Fy__rl) + ((Lr * (h__Gs - z__static) * ms - Lr * (h__Gs - z__static) * m + is__xz) * Fy__rr) - ((AM__fl + AM__fr + AM__rl + AM__rr) * (h__Gs - z__static) * (ms - m))) * ms * z - ((h__Gs - z__static) * u * (z__static * (h__Gs - z__static) * ms ^ 2 - m * z__static * (h__Gs - z__static) * ms + is__xx * m) * ms * Omega * mu) - (is__xz * (-iwa__f * omega__fl - iwa__f * omega__fr + (is__xx - is__yy + is__zz) * mu__dot - iwa__r * (omega__rl + omega__rr)) * m * Omega) + (((z__static * Lf * (h__Gs - z__static) * ms ^ 2 - z__static * (Lf * (h__Gs - z__static) * m + is__xz) * ms + m * (is__xx * Lf - is__xz * Rf + h__Gs * is__xz)) * Fx__fl) + (Wf * (z__static * (h__Gs - z__static) * ms ^ 2 - m * z__static * (h__Gs - z__static) * ms + is__xx * m) * Fy__fl) / 0.2e1 + (is__xz * m * Tw__fl)) * delta__fl + (((z__static * Lf * (h__Gs - z__static) * ms ^ 2 - z__static * (Lf * (h__Gs - z__static) * m + is__xz) * ms + m * (is__xx * Lf - is__xz * Rf + h__Gs * is__xz)) * Fx__fr) - (Wf * (z__static * (h__Gs - z__static) * ms ^ 2 - m * z__static * (h__Gs - z__static) * ms + is__xx * m) * Fy__fr) / 0.2e1 + (is__xz * m * Tw__fr)) * delta__fr - (Wf * (z__static * (h__Gs - z__static) * ms ^ 2 - m * z__static * (h__Gs - z__static) * ms + is__xx * m) * Fx__fl) / 0.2e1 + (Wf * (z__static * (h__Gs - z__static) * ms ^ 2 - m * z__static * (h__Gs - z__static) * ms + is__xx * m) * Fx__fr) / 0.2e1 + ((z__static * Lf * (h__Gs - z__static) * ms ^ 2 - z__static * (Lf * (h__Gs - z__static) * m + is__xz) * ms + m * (is__xx * Lf + h__Gs * is__xz)) * Fy__fl) + ((z__static * Lf * (h__Gs - z__static) * ms ^ 2 - z__static * (Lf * (h__Gs - z__static) * m + is__xz) * ms + m * (is__xx * Lf + h__Gs * is__xz)) * Fy__fr) - (Wr * (z__static * (h__Gs - z__static) * ms ^ 2 - m * z__static * (h__Gs - z__static) * ms + is__xx * m) * Fx__rl) / 0.2e1 + (Wr * (z__static * (h__Gs - z__static) * ms ^ 2 - m * z__static * (h__Gs - z__static) * ms + is__xx * m) * Fx__rr) / 0.2e1 + (is__xz * m * Fz__fl * Wf) / 0.2e1 - (is__xz * m * Fz__fr * Wf) / 0.2e1 + (is__xz * m * Fz__rl * Wr) / 0.2e1 - (is__xz * m * Fz__rr * Wr) / 0.2e1 + ((-Lr * z__static * (h__Gs - z__static) * ms ^ 2 + z__static * (Lr * (h__Gs - z__static) * m - is__xz) * ms + m * (-Lr * is__xx + h__Gs * is__xz)) * Fy__rl) + ((-Lr * z__static * (h__Gs - z__static) * ms ^ 2 + z__static * (Lr * (h__Gs - z__static) * m - is__xz) * ms + m * (-Lr * is__xx + h__Gs * is__xz)) * Fy__rr) + ((AM__fl + AM__fr + AM__rl + AM__rr) * (z__static * (h__Gs - z__static) * ms ^ 2 - m * z__static * (h__Gs - z__static) * ms + is__xx * m))) * (ms * (h__Gs - z__static) * (ms - m) * z - z__static * (h__Gs - z__static) * ms ^ 2 + m * z__static * (h__Gs - z__static) * ms - m * (is__yy - is__zz)) * phi - 0.2e1 * (((-ms * Omega ^ 2 * (h__Gs - z__static) * (ms - m) * mu + 2 * ms * phi__dot * (h__Gs - z__static) * (ms - m) * Omega + ms * Fy__fl * delta__fl + ms * Fy__fr * delta__fr - ms * Fx__fl - ms * Fx__fr - ms * Fx__rl - ms * Fx__rr + FAxc * (ms - m)) * z) + (((z__static * (h__Gs - z__static) * ms ^ 2 - m * z__static * (h__Gs - z__static) * ms + m * (is__xx - is__zz)) * Omega ^ 2 + m * (h__Gs - z__static) * (-m * g + g * ms - FAz__f - FAz__r + Fz__fl + Fz__fr + Fz__rl + Fz__rr)) * mu) + (i__xz * m * Omega ^ 2) + ((iwa__f * m * delta__fl * omega__fl) + (iwa__f * m * delta__fr * omega__fr) - 0.2e1 * ((z__static * (h__Gs - z__static) * ms ^ 2) - (m * z__static * (h__Gs - z__static) * ms) + (m * (is__xx + is__yy - is__zz)) / 0.2e1) * phi__dot) * Omega - (Fy__fl * (-m * h__Gs + z__static * ms) * delta__fl) - (Fy__fr * (-m * h__Gs + z__static * ms) * delta__fr) + ((z__static * ms - m * (h__Gs - Rf)) * Fx__fl) + ((z__static * ms - m * (h__Gs - Rf)) * Fx__fr) + ((z__static * ms - m * (h__Gs - Rr)) * Fx__rl) + ((z__static * ms - m * (h__Gs - Rr)) * Fx__rr) - (m * Lf * Fz__fl) - (m * Lf * Fz__fr) + (m * Fz__rl * Lr) + (m * Fz__rr * Lr) + (m * FAz__f * Lf) - (m * FAz__r * Lr) + ((m * h__Gs - z__static * ms) * FAxc) - (m * (Tw__fl + Tw__fr + Tw__rl + Tw__rr))) * (ms * (is__xz * mu + i__zz) * (h__Gs - z__static) * (ms - m) * z - is__xz * (z__static * (h__Gs - z__static) * ms ^ 2 - m * z__static * (h__Gs - z__static) * ms + m * (is__xx + is__zz)) * mu - i__zz * z__static * (h__Gs - z__static) * ms ^ 2 + i__zz * m * z__static * (h__Gs - z__static) * ms + m * (i__xz * is__xz - i__zz * is__xx))) / (0.2e1 * ((h__Gs - z__static) ^ 2) * (ms * (h__Gs - z__static) * (ms - m) * z - z__static * (h__Gs - z__static) * ms ^ 2 + m * z__static * (h__Gs - z__static) * ms - is__xx * m) * is__zz * (ms ^ 2) * phi ^ 2 + (2 * (ms * (h__Gs - z__static) * (ms - m) * z - z__static * (h__Gs - z__static) * ms ^ 2 + m * z__static * (h__Gs - z__static) * ms - is__yy * m) * (ms * (is__xz * mu + i__zz) * (h__Gs - z__static) * (ms - m) * z - is__xz * (z__static * (h__Gs - z__static) * ms ^ 2 - m * z__static * (h__Gs - z__static) * ms + m * (is__xx + is__zz)) * mu - i__zz * z__static * (h__Gs - z__static) * ms ^ 2 + i__zz * m * z__static * (h__Gs - z__static) * ms + m * (i__xz * is__xz - i__zz * is__xx))));
Omega_Dot    = (-0.2e1 * (h__Gs - z__static) * (ms - m) * ((h__Gs - z__static) * (-is__xz * (ms - m) * Omega ^ 2 + ms * v * (h__Gs - z__static) * (ms - m) * Omega - ms * (-delta__fl * Fy__fl - delta__fr * Fy__fr + Fx__fl + Fx__fr + Fx__rl + Fx__rr) * (h__Gs - z__static)) * phi + ms * u * mu * (h__Gs - z__static) ^ 2 * (ms - m) * Omega + ((-Lf * (h__Gs - z__static) * ms + h__Gs * m * Lf - m * z__static * Lf + is__xz) * Fx__fl - Fy__fl * Wf * (h__Gs - z__static) * (ms - m) / 0.2e1) * delta__fl + ((-Lf * (h__Gs - z__static) * ms + h__Gs * m * Lf - m * z__static * Lf + is__xz) * Fx__fr + Fy__fr * Wf * (h__Gs - z__static) * (ms - m) / 0.2e1) * delta__fr + Wf * (h__Gs - z__static) * (ms - m) * Fx__fl / 0.2e1 - Wf * (h__Gs - z__static) * (ms - m) * Fx__fr / 0.2e1 + (-Lf * (h__Gs - z__static) * ms + h__Gs * m * Lf - m * z__static * Lf + is__xz) * Fy__fl + (-Lf * (h__Gs - z__static) * ms + h__Gs * m * Lf - m * z__static * Lf + is__xz) * Fy__fr + Wr * (h__Gs - z__static) * (ms - m) * Fx__rl / 0.2e1 - Wr * (h__Gs - z__static) * (ms - m) * Fx__rr / 0.2e1 + (Lr * (h__Gs - z__static) * ms - h__Gs * m * Lr + m * z__static * Lr + is__xz) * Fy__rl + (Lr * (h__Gs - z__static) * ms - h__Gs * m * Lr + m * z__static * Lr + is__xz) * Fy__rr - (AM__fl + AM__fr + AM__rl + AM__rr) * (h__Gs - z__static) * (ms - m)) * ms ^ 2 * z ^ 2 - 0.2e1 * ((h__Gs - z__static) * ((ms ^ 2 * (h__Gs - z__static) ^ 2 * (is__xx - is__yy - is__zz) * mu + ((-i__xz + 0.2e1 * is__xz) * z__static + h__Gs * i__xz) * (h__Gs - z__static) * ms ^ 2 - 0.2e1 * is__xz * m * z__static * (h__Gs - z__static) * ms + 0.2e1 * is__xz * (is__yy - is__zz / 0.2e1) * m) * (ms - m) * Omega ^ 2 - 0.2e1 * (h__Gs - z__static) * (-ms * iwa__f * omega__fl * (h__Gs - z__static) * delta__fl / 0.2e1 - ms * iwa__f * omega__fr * (h__Gs - z__static) * delta__fr / 0.2e1 + (z__static * (h__Gs - z__static) * ms ^ 2 - m * z__static * (h__Gs - z__static) * ms + m * (is__xx + is__yy) / 0.2e1) * v + ms * phi__dot * (is__xx - is__yy - is__zz) * (h__Gs - z__static) / 0.2e1) * (ms - m) * ms * Omega + (ms ^ 2 * (h__Gs - z__static) ^ 2 * (ms - m) * (-m * g + g * ms - FAz__f - FAz__r + Fz__fl + Fz__fr + Fz__rl + Fz__rr) * mu + Fy__fl * ((h__Gs - z__static) * (h__Gs - 0.2e1 * z__static) * ms ^ 2 + (-h__Gs ^ 2 * m + 0.3e1 * h__Gs * m * z__static - 0.2e1 * m * z__static ^ 2 + is__yy) * ms - m * (is__xx + is__yy)) * ms * delta__fl + Fy__fr * ((h__Gs - z__static) * (h__Gs - 0.2e1 * z__static) * ms ^ 2 + (-h__Gs ^ 2 * m + 0.3e1 * h__Gs * m * z__static - 0.2e1 * m * z__static ^ 2 + is__yy) * ms - m * (is__xx + is__yy)) * ms * delta__fr - ((h__Gs - z__static) * (h__Gs - 0.2e1 * z__static - Rf) * ms ^ 2 + (-0.2e1 * m * z__static ^ 2 + 0.3e1 * (h__Gs - Rf / 0.3e1) * m * z__static - h__Gs * (h__Gs - Rf) * m + is__yy) * ms - m * (is__xx + is__yy)) * ms * Fx__fl - ((h__Gs - z__static) * (h__Gs - 0.2e1 * z__static - Rf) * ms ^ 2 + (-0.2e1 * m * z__static ^ 2 + 0.3e1 * (h__Gs - Rf / 0.3e1) * m * z__static - h__Gs * (h__Gs - Rf) * m + is__yy) * ms - m * (is__xx + is__yy)) * ms * Fx__fr - ((h__Gs - z__static) * (h__Gs - 0.2e1 * z__static - Rr) * ms ^ 2 + (-0.2e1 * m * z__static ^ 2 + 0.3e1 * (h__Gs - Rr / 0.3e1) * m * z__static - h__Gs * (h__Gs - Rr) * m + is__yy) * ms - m * (is__xx + is__yy)) * ms * Fx__rl - ((h__Gs - z__static) * (h__Gs - 0.2e1 * z__static - Rr) * ms ^ 2 + (-0.2e1 * m * z__static ^ 2 + 0.3e1 * (h__Gs - Rr / 0.3e1) * m * z__static - h__Gs * (h__Gs - Rr) * m + is__yy) * ms - m * (is__xx + is__yy)) * ms * Fx__rr + ((-Lf * (h__Gs - z__static) * ms ^ 2 + is__xz * m) * Fz__fl + (-Lf * (h__Gs - z__static) * ms ^ 2 + is__xz * m) * Fz__fr + (Lr * (h__Gs - z__static) * ms ^ 2 + is__xz * m) * Fz__rl + (Lr * (h__Gs - z__static) * ms ^ 2 + is__xz * m) * Fz__rr + (Lf * (h__Gs - z__static) * ms ^ 2 - is__xz * m) * FAz__f + (-Lr * (h__Gs - z__static) * ms ^ 2 - is__xz * m) * FAz__r + ((h__Gs - z__static) ^ 2 * ms + is__yy) * ms * FAxc - ms ^ 2 * (h__Gs - z__static) * Tw__fl - ms ^ 2 * (h__Gs - z__static) * Tw__fr - ms ^ 2 * (h__Gs - z__static) * Tw__rl - ms ^ 2 * (h__Gs - z__static) * Tw__rr + g * is__xz * m * (ms - m)) * (ms - m)) * (h__Gs - z__static)) * phi - 0.2e1 * ((z__static * (h__Gs - z__static) * ms ^ 2 - m * z__static * (h__Gs - z__static) * ms + m * (is__xx + is__yy) / 0.2e1) * (h__Gs - z__static) * u * ms * mu + is__xz * (-iwa__f * omega__fl - iwa__f * omega__fr + (is__xx - is__yy + is__zz) * mu__dot - iwa__r * (omega__rl + omega__rr)) * m / 0.2e1) * (h__Gs - z__static) * (ms - m) * Omega + ((0.2e1 * z__static * Lf * (h__Gs - z__static) ^ 2 * ms ^ 3 - 0.4e1 * (h__Gs - z__static) * (h__Gs * m * Lf - m * z__static * Lf + is__xz / 0.2e1) * z__static * ms ^ 2 + (h__Gs - z__static) * m * (-0.2e1 * m * z__static ^ 2 * Lf + (0.2e1 * h__Gs * m * Lf + 0.2e1 * is__xz) * z__static + h__Gs * is__xz - is__xz * Rf + Lf * (is__xx + is__yy)) * ms - (-(h__Gs * is__xz - is__xz * Rf + Lf * (is__xx + is__yy)) * m * z__static + h__Gs * (h__Gs * is__xz - is__xz * Rf + Lf * (is__xx + is__yy)) * m + is__yy * is__xz) * m) * Fx__fl + (h__Gs - z__static) * ((z__static * (h__Gs - z__static) * ms ^ 2 - m * z__static * (h__Gs - z__static) * ms + m * (is__xx + is__yy) / 0.2e1) * Wf * Fy__fl + is__xz * m * Tw__fl) * (ms - m)) * delta__fl + ((0.2e1 * z__static * Lf * (h__Gs - z__static) ^ 2 * ms ^ 3 - 0.4e1 * (h__Gs - z__static) * (h__Gs * m * Lf - m * z__static * Lf + is__xz / 0.2e1) * z__static * ms ^ 2 + (h__Gs - z__static) * m * (-0.2e1 * m * z__static ^ 2 * Lf + (0.2e1 * h__Gs * m * Lf + 0.2e1 * is__xz) * z__static + h__Gs * is__xz - is__xz * Rf + Lf * (is__xx + is__yy)) * ms - (-(h__Gs * is__xz - is__xz * Rf + Lf * (is__xx + is__yy)) * m * z__static + h__Gs * (h__Gs * is__xz - is__xz * Rf + Lf * (is__xx + is__yy)) * m + is__yy * is__xz) * m) * Fx__fr - (h__Gs - z__static) * ((z__static * (h__Gs - z__static) * ms ^ 2 - m * z__static * (h__Gs - z__static) * ms + m * (is__xx + is__yy) / 0.2e1) * Wf * Fy__fr - is__xz * m * Tw__fr) * (ms - m)) * delta__fr - (z__static * (h__Gs - z__static) * ms ^ 2 - m * z__static * (h__Gs - z__static) * ms + m * (is__xx + is__yy) / 0.2e1) * (h__Gs - z__static) * Wf * (ms - m) * Fx__fl + (z__static * (h__Gs - z__static) * ms ^ 2 - m * z__static * (h__Gs - z__static) * ms + m * (is__xx + is__yy) / 0.2e1) * (h__Gs - z__static) * Wf * (ms - m) * Fx__fr + (0.2e1 * z__static * Lf * (h__Gs - z__static) ^ 2 * ms ^ 3 - 0.4e1 * (h__Gs - z__static) * (h__Gs * m * Lf - m * z__static * Lf + is__xz / 0.2e1) * z__static * ms ^ 2 + (h__Gs - z__static) * (-0.2e1 * m * z__static ^ 2 * Lf + (0.2e1 * h__Gs * m * Lf + 0.2e1 * is__xz) * z__static + h__Gs * is__xz + Lf * (is__xx + is__yy)) * m * ms - m * (-(h__Gs * is__xz + Lf * (is__xx + is__yy)) * m * z__static + h__Gs * (h__Gs * is__xz + Lf * (is__xx + is__yy)) * m + is__yy * is__xz)) * Fy__fl + (0.2e1 * z__static * Lf * (h__Gs - z__static) ^ 2 * ms ^ 3 - 0.4e1 * (h__Gs - z__static) * (h__Gs * m * Lf - m * z__static * Lf + is__xz / 0.2e1) * z__static * ms ^ 2 + (h__Gs - z__static) * (-0.2e1 * m * z__static ^ 2 * Lf + (0.2e1 * h__Gs * m * Lf + 0.2e1 * is__xz) * z__static + h__Gs * is__xz + Lf * (is__xx + is__yy)) * m * ms - m * (-(h__Gs * is__xz + Lf * (is__xx + is__yy)) * m * z__static + h__Gs * (h__Gs * is__xz + Lf * (is__xx + is__yy)) * m + is__yy * is__xz)) * Fy__fr - (z__static * (h__Gs - z__static) * ms ^ 2 - m * z__static * (h__Gs - z__static) * ms + m * (is__xx + is__yy) / 0.2e1) * (h__Gs - z__static) * Wr * (ms - m) * Fx__rl + (z__static * (h__Gs - z__static) * ms ^ 2 - m * z__static * (h__Gs - z__static) * ms + m * (is__xx + is__yy) / 0.2e1) * (h__Gs - z__static) * Wr * (ms - m) * Fx__rr + is__xz * m * Wf * (h__Gs - z__static) * (ms - m) * Fz__fl / 0.2e1 - is__xz * m * Wf * (h__Gs - z__static) * (ms - m) * Fz__fr / 0.2e1 + is__xz * m * Wr * (h__Gs - z__static) * (ms - m) * Fz__rl / 0.2e1 - is__xz * m * Wr * (h__Gs - z__static) * (ms - m) * Fz__rr / 0.2e1 + (-0.2e1 * Lr * z__static * (h__Gs - z__static) ^ 2 * ms ^ 3 + 0.4e1 * (h__Gs - z__static) * z__static * (h__Gs * m * Lr - m * z__static * Lr - is__xz / 0.2e1) * ms ^ 2 + (h__Gs - z__static) * m * (0.2e1 * m * z__static ^ 2 * Lr + (-0.2e1 * h__Gs * m * Lr + 0.2e1 * is__xz) * z__static + h__Gs * is__xz - Lr * (is__xx + is__yy)) * ms - m * (-(h__Gs * is__xz - Lr * (is__xx + is__yy)) * m * z__static + h__Gs * (h__Gs * is__xz - Lr * (is__xx + is__yy)) * m + is__yy * is__xz)) * Fy__rl + (-0.2e1 * Lr * z__static * (h__Gs - z__static) ^ 2 * ms ^ 3 + 0.4e1 * (h__Gs - z__static) * z__static * (h__Gs * m * Lr - m * z__static * Lr - is__xz / 0.2e1) * ms ^ 2 + (h__Gs - z__static) * m * (0.2e1 * m * z__static ^ 2 * Lr + (-0.2e1 * h__Gs * m * Lr + 0.2e1 * is__xz) * z__static + h__Gs * is__xz - Lr * (is__xx + is__yy)) * ms - m * (-(h__Gs * is__xz - Lr * (is__xx + is__yy)) * m * z__static + h__Gs * (h__Gs * is__xz - Lr * (is__xx + is__yy)) * m + is__yy * is__xz)) * Fy__rr + 0.2e1 * (z__static * (h__Gs - z__static) * ms ^ 2 - m * z__static * (h__Gs - z__static) * ms + m * (is__xx + is__yy) / 0.2e1) * (h__Gs - z__static) * (ms - m) * (AM__fl + AM__fr + AM__rl + AM__rr)) * ms * z + ((0.2e1 * (is__xx - is__yy - is__zz) * (h__Gs - z__static) ^ 2 * (z__static * (h__Gs - z__static) * ms ^ 2 - m * z__static * (h__Gs - z__static) * ms + is__xx * m) * ms ^ 2 * mu + 0.2e1 * (h__Gs - z__static) ^ 2 * z__static * ((-i__xz + is__xz) * z__static + h__Gs * i__xz) * ms ^ 4 - 0.2e1 * ((-i__xz + 0.2e1 * is__xz) * z__static + h__Gs * i__xz) * (h__Gs - z__static) ^ 2 * z__static * m * ms ^ 3 + 0.2e1 * (h__Gs - z__static) * m * (-is__xz * m * z__static ^ 3 + h__Gs * is__xz * m * z__static ^ 2 + ((0.2e1 * is__yy - is__zz) * is__xz - i__xz * is__xx) * z__static + h__Gs * i__xz * is__xx) * ms ^ 2 - 0.4e1 * is__xz * (h__Gs - z__static) * z__static * (is__yy - is__zz / 0.2e1) * m ^ 2 * ms + 0.2e1 * is__xz * is__yy * m ^ 2 * (is__yy - is__zz)) * Omega ^ 2 - 0.2e1 * (h__Gs - z__static) * (-ms * iwa__f * omega__fl * (h__Gs - z__static) * delta__fl - ms * iwa__f * omega__fr * (h__Gs - z__static) * delta__fr + (z__static * (h__Gs - z__static) * ms ^ 2 - m * z__static * (h__Gs - z__static) * ms + is__yy * m) * v + ms * phi__dot * (is__xx - is__yy - is__zz) * (h__Gs - z__static)) * (z__static * (h__Gs - z__static) * ms ^ 2 - m * z__static * (h__Gs - z__static) * ms + is__xx * m) * ms * Omega + 0.2e1 * ((h__Gs - z__static) ^ 2 * (z__static * (h__Gs - z__static) * ms ^ 2 - m * z__static * (h__Gs - z__static) * ms + is__xx * m) * ms ^ 2 * (-m * g + g * ms - FAz__f - FAz__r + Fz__fl + Fz__fr + Fz__rl + Fz__rr) * mu + ((h__Gs - z__static) ^ 2 * ms + is__yy) * Fy__fl * (z__static * (h__Gs - z__static) * ms ^ 2 - m * z__static * (h__Gs - z__static) * ms + is__xx * m) * ms * delta__fl + ((h__Gs - z__static) ^ 2 * ms + is__yy) * Fy__fr * (z__static * (h__Gs - z__static) * ms ^ 2 - m * z__static * (h__Gs - z__static) * ms + is__xx * m) * ms * delta__fr - ((h__Gs - z__static) * (h__Gs - z__static - Rf) * ms + is__yy) * (z__static * (h__Gs - z__static) * ms ^ 2 - m * z__static * (h__Gs - z__static) * ms + is__xx * m) * ms * Fx__fl - ((h__Gs - z__static) * (h__Gs - z__static - Rf) * ms + is__yy) * (z__static * (h__Gs - z__static) * ms ^ 2 - m * z__static * (h__Gs - z__static) * ms + is__xx * m) * ms * Fx__fr - ((h__Gs - z__static) * (h__Gs - z__static - Rr) * ms + is__yy) * (z__static * (h__Gs - z__static) * ms ^ 2 - m * z__static * (h__Gs - z__static) * ms + is__xx * m) * ms * Fx__rl - ((h__Gs - z__static) * (h__Gs - z__static - Rr) * ms + is__yy) * (z__static * (h__Gs - z__static) * ms ^ 2 - m * z__static * (h__Gs - z__static) * ms + is__xx * m) * ms * Fx__rr + (-z__static * Lf * (h__Gs - z__static) ^ 2 * ms ^ 4 + m * z__static * Lf * (h__Gs - z__static) ^ 2 * ms ^ 3 - m * (is__xx * Lf - is__xz * z__static) * (h__Gs - z__static) * ms ^ 2 - is__xz * m ^ 2 * z__static * (h__Gs - z__static) * ms + is__xz * is__yy * m ^ 2) * Fz__fl + (-z__static * Lf * (h__Gs - z__static) ^ 2 * ms ^ 4 + m * z__static * Lf * (h__Gs - z__static) ^ 2 * ms ^ 3 - m * (is__xx * Lf - is__xz * z__static) * (h__Gs - z__static) * ms ^ 2 - is__xz * m ^ 2 * z__static * (h__Gs - z__static) * ms + is__xz * is__yy * m ^ 2) * Fz__fr + (Lr * z__static * (h__Gs - z__static) ^ 2 * ms ^ 4 - m * z__static * Lr * (h__Gs - z__static) ^ 2 * ms ^ 3 + m * (Lr * is__xx + is__xz * z__static) * (h__Gs - z__static) * ms ^ 2 - is__xz * m ^ 2 * z__static * (h__Gs - z__static) * ms + is__xz * is__yy * m ^ 2) * Fz__rl + (Lr * z__static * (h__Gs - z__static) ^ 2 * ms ^ 4 - m * z__static * Lr * (h__Gs - z__static) ^ 2 * ms ^ 3 + m * (Lr * is__xx + is__xz * z__static) * (h__Gs - z__static) * ms ^ 2 - is__xz * m ^ 2 * z__static * (h__Gs - z__static) * ms + is__xz * is__yy * m ^ 2) * Fz__rr + (z__static * Lf * (h__Gs - z__static) ^ 2 * ms ^ 4 - m * z__static * Lf * (h__Gs - z__static) ^ 2 * ms ^ 3 + m * (is__xx * Lf - is__xz * z__static) * (h__Gs - z__static) * ms ^ 2 + is__xz * m ^ 2 * z__static * (h__Gs - z__static) * ms - is__xz * is__yy * m ^ 2) * FAz__f + (-Lr * z__static * (h__Gs - z__static) ^ 2 * ms ^ 4 + m * z__static * Lr * (h__Gs - z__static) ^ 2 * ms ^ 3 - m * (Lr * is__xx + is__xz * z__static) * (h__Gs - z__static) * ms ^ 2 + is__xz * m ^ 2 * z__static * (h__Gs - z__static) * ms - is__xz * is__yy * m ^ 2) * FAz__r + ((h__Gs - z__static) ^ 2 * ms + is__yy) * (z__static * (h__Gs - z__static) * ms ^ 2 - m * z__static * (h__Gs - z__static) * ms + is__xx * m) * ms * FAxc - (h__Gs - z__static) * (z__static * (h__Gs - z__static) * ms ^ 2 - m * z__static * (h__Gs - z__static) * ms + is__xx * m) * ms ^ 2 * Tw__fl - (h__Gs - z__static) * (z__static * (h__Gs - z__static) * ms ^ 2 - m * z__static * (h__Gs - z__static) * ms + is__xx * m) * ms ^ 2 * Tw__fr - (h__Gs - z__static) * (z__static * (h__Gs - z__static) * ms ^ 2 - m * z__static * (h__Gs - z__static) * ms + is__xx * m) * ms ^ 2 * Tw__rl - (h__Gs - z__static) * (z__static * (h__Gs - z__static) * ms ^ 2 - m * z__static * (h__Gs - z__static) * ms + is__xx * m) * ms ^ 2 * Tw__rr + is__xz * (ms - m) * m * (z__static * (h__Gs - z__static) * ms ^ 2 - m * z__static * (h__Gs - z__static) * ms + is__yy * m) * g) * (h__Gs - z__static)) * phi - 0.2e1 * (((h__Gs - z__static) * u * (z__static * (h__Gs - z__static) * ms ^ 2 - m * z__static * (h__Gs - z__static) * ms + is__xx * m) * ms * mu + is__xz * (-iwa__f * omega__fl - iwa__f * omega__fr + (is__xx - is__yy + is__zz) * mu__dot - iwa__r * (omega__rl + omega__rr)) * m) * Omega + ((-z__static * Lf * (h__Gs - z__static) * ms ^ 2 + z__static * (h__Gs * m * Lf - m * z__static * Lf + is__xz) * ms - m * (is__xx * Lf - is__xz * Rf + h__Gs * is__xz)) * Fx__fl - Wf * (z__static * (h__Gs - z__static) * ms ^ 2 - m * z__static * (h__Gs - z__static) * ms + is__xx * m) * Fy__fl / 0.2e1 - is__xz * m * Tw__fl) * delta__fl + ((-z__static * Lf * (h__Gs - z__static) * ms ^ 2 + z__static * (h__Gs * m * Lf - m * z__static * Lf + is__xz) * ms - m * (is__xx * Lf - is__xz * Rf + h__Gs * is__xz)) * Fx__fr + Wf * (z__static * (h__Gs - z__static) * ms ^ 2 - m * z__static * (h__Gs - z__static) * ms + is__xx * m) * Fy__fr / 0.2e1 - is__xz * m * Tw__fr) * delta__fr + Wf * (z__static * (h__Gs - z__static) * ms ^ 2 - m * z__static * (h__Gs - z__static) * ms + is__xx * m) * Fx__fl / 0.2e1 - Wf * (z__static * (h__Gs - z__static) * ms ^ 2 - m * z__static * (h__Gs - z__static) * ms + is__xx * m) * Fx__fr / 0.2e1 + (-z__static * Lf * (h__Gs - z__static) * ms ^ 2 + z__static * (h__Gs * m * Lf - m * z__static * Lf + is__xz) * ms - m * (is__xx * Lf + h__Gs * is__xz)) * Fy__fl + (-z__static * Lf * (h__Gs - z__static) * ms ^ 2 + z__static * (h__Gs * m * Lf - m * z__static * Lf + is__xz) * ms - m * (is__xx * Lf + h__Gs * is__xz)) * Fy__fr + Wr * (z__static * (h__Gs - z__static) * ms ^ 2 - m * z__static * (h__Gs - z__static) * ms + is__xx * m) * Fx__rl / 0.2e1 - Wr * (z__static * (h__Gs - z__static) * ms ^ 2 - m * z__static * (h__Gs - z__static) * ms + is__xx * m) * Fx__rr / 0.2e1 - is__xz * m * Fz__fl * Wf / 0.2e1 + is__xz * m * Fz__fr * Wf / 0.2e1 - is__xz * m * Fz__rl * Wr / 0.2e1 + is__xz * m * Fz__rr * Wr / 0.2e1 + (Lr * z__static * (h__Gs - z__static) * ms ^ 2 - z__static * (h__Gs * m * Lr - m * z__static * Lr - is__xz) * ms - m * (-Lr * is__xx + h__Gs * is__xz)) * Fy__rl + (Lr * z__static * (h__Gs - z__static) * ms ^ 2 - z__static * (h__Gs * m * Lr - m * z__static * Lr - is__xz) * ms - m * (-Lr * is__xx + h__Gs * is__xz)) * Fy__rr - (AM__fl + AM__fr + AM__rl + AM__rr) * (z__static * (h__Gs - z__static) * ms ^ 2 - m * z__static * (h__Gs - z__static) * ms + is__xx * m)) * (z__static * (h__Gs - z__static) * ms ^ 2 - m * z__static * (h__Gs - z__static) * ms + is__yy * m)) / (0.2e1 * ms ^ 2 * (h__Gs - z__static) ^ 2 * (ms - m) ^ 2 * (is__xz * mu + i__zz) * z ^ 2 + 0.2e1 * (ms ^ 2 * is__zz * (h__Gs - z__static) ^ 2 * phi ^ 2 - 0.2e1 * is__xz * (z__static * (h__Gs - z__static) * ms ^ 2 - m * z__static * (h__Gs - z__static) * ms + m * (is__xx + is__yy + is__zz) / 0.2e1) * mu - 0.2e1 * i__zz * z__static * (h__Gs - z__static) * ms ^ 2 + 0.2e1 * i__zz * m * z__static * (h__Gs - z__static) * ms + (i__xz * is__xz - i__zz * (is__xx + is__yy)) * m) * (h__Gs - z__static) * (ms - m) * ms * z - 0.2e1 * (h__Gs - z__static) ^ 2 * is__zz * (z__static * (h__Gs - z__static) * ms ^ 2 - m * z__static * (h__Gs - z__static) * ms + is__xx * m) * ms ^ 2 * phi ^ 2 + 0.2e1 * (is__xz * (z__static * (h__Gs - z__static) * ms ^ 2 - m * z__static * (h__Gs - z__static) * ms + m * (is__xx + is__zz)) * mu + i__zz * z__static * (h__Gs - z__static) * ms ^ 2 - i__zz * m * z__static * (h__Gs - z__static) * ms - m * (i__xz * is__xz - i__zz * is__xx)) * (z__static * (h__Gs - z__static) * ms ^ 2 - m * z__static * (h__Gs - z__static) * ms + is__yy * m));
% Steering wheel first order dynamics
delta_Dot    = (-delta * tau__D + delta_req) / tau__D / tau__H;
% Side slip angle first order dynamics
alpha_rr_Dot = 0.2e1 * ((-alpha__rr * Wr / 0.2e1 + Lr) * Omega - u * alpha__rr - v) * u / ly / (Omega * Wr + 0.2e1 * u);
alpha_rl_Dot = -0.2e1 * u * ((alpha__rl * Wr / 0.2e1 + Lr) * Omega - u * alpha__rl - v) / ly / (Omega * Wr - 0.2e1 * u);
alpha_fr_Dot = 0.4e1 * u * (((Lf ^ 2 + Wf ^ 2 / 0.4e1) * delta__fr - Wf * (alpha__fr * Wf / 0.2e1 + Lf) / 0.2e1) * Omega ^ 2 + ((-alpha__fr * Wf + delta__fr * Wf - Lf) * u - v * Wf / 0.2e1) * Omega - u * ((alpha__fr - delta__fr) * u + v)) / ly / (Omega * Wf + 0.2e1 * u) ^ 2;
alpha_fl_Dot = 0.4e1 * u * (((Lf ^ 2 + Wf ^ 2 / 0.4e1) * delta__fl + Wf * (-alpha__fl * Wf / 0.2e1 + Lf) / 0.2e1) * Omega ^ 2 + ((alpha__fl * Wf - delta__fl * Wf - Lf) * u + v * Wf / 0.2e1) * Omega - u * ((alpha__fl - delta__fl) * u + v)) / ly / (Omega * Wf - 0.2e1 * u) ^ 2;
% Longitudinal slip first order dynamics
kappa_rr_Dot = -abs(u) * (kappa__rr - kappa__rr_ss) / lx;
kappa_rl_Dot = -abs(u) * (kappa__rl - kappa__rl_ss) / lx;
kappa_fr_Dot = -abs(u) * (kappa__fr - kappa__fr_ss) / lx;
kappa_fl_Dot = -abs(u) * (kappa__fl - kappa__fl_ss) / lx;
% Wheel spin dynamics
omega_rr_Dot = (-Fx__rr * Rr + Tw__rr) / iwa__r;
omega_rl_Dot = (-Fx__rl * Rr + Tw__rl) / iwa__r;
omega_fr_Dot = (-Fx__fr * Rf + Tw__fr) / iwa__f;
omega_fl_Dot = (-Fx__fl * Rf + Tw__fl) / iwa__f;
% Motor dynamics
Tm_Dot       = (Tm_req - Tm) / tau_mot;
% Braking system dynamics 
Tb_Dot       = (Tb_req - Tb) / tau_br;
% Equations for first order reduction
z_Dot        = z__dot;
phi_Dot      = phi__dot;
mu_Dot       = mu__dot;

% Collect states derivatives in the dX vector
dX(1)  = u_Dot;
dX(2)  = v_Dot;
dX(3)  = z_Dot;
dX(4)  = Omega_Dot;
dX(5)  = phi_Dot;
dX(6)  = mu_Dot;
dX(7)  = delta_Dot;
dX(8)  = alpha_rr_Dot;
dX(9)  = alpha_rl_Dot;
dX(10) = alpha_fr_Dot;
dX(11) = alpha_fl_Dot;
dX(12) = kappa_rr_Dot;
dX(13) = kappa_rl_Dot;
dX(14) = kappa_fr_Dot;
dX(15) = kappa_fl_Dot;
dX(16) = omega_rr_Dot;
dX(17) = omega_rl_Dot;
dX(18) = omega_fr_Dot;
dX(19) = omega_fl_Dot;
dX(20) = z_DDot;
dX(21) = phi_DDot;
dX(22) = mu_DDot;
dX(23) = Tm_Dot;
dX(24) = Tb_Dot;
  

% ----------------------------------------------------------------
%% SAVE USEFUL EXTRA PARAMETERS
% ----------------------------------------------------------------

extra_params(1)  = Tw__rr;
extra_params(2)  = Tw__rl;
extra_params(3)  = Tw__fr;
extra_params(4)  = Tw__fl;
extra_params(5)  = Fx__rr;
extra_params(6)  = Fx__rl;
extra_params(7)  = Fx__fr;
extra_params(8)  = Fx__fl;
extra_params(9)  = Fy__rr;
extra_params(10) = Fy__rl;
extra_params(11) = Fy__fr;
extra_params(12) = Fy__fl;
extra_params(13) = Fz__rr;
extra_params(14) = Fz__rl;
extra_params(15) = Fz__fr;
extra_params(16) = Fz__fl;
extra_params(17) = AM__rr;
extra_params(18) = AM__rl;
extra_params(19) = AM__fr;
extra_params(20) = AM__fl;
extra_params(21) = gamma__rr;
extra_params(22) = gamma__rl;
extra_params(23) = gamma__fr;
extra_params(24) = gamma__fl;
extra_params(25) = delta__fr;
extra_params(26) = delta__fl;

end
